simulink library "ddm"  (R2021b)
settings: Solver=VariableStepAuto  StartTime=0.0  StopTime=10.0  RelTol=1e-3
undefined symbols (not defined in the file or in its folder): ADDM_FrTMTqDev_X_Nm, ADDM_RrTMTqDev_X_Nm, ENUM_ADASACCSTA_ERROR, ENUM_ADASACCSTA_OFF, ENUM_ADASACCSTA_STANDBY, ENUM_ALLOWMOV_ALLOWREADY, ENUM_APS, ENUM_BRKSTA_ERROR, ENUM_BRKSTA_OFF, ENUM_BRKSTA_ON, ENUM_BRKSW_INVALID, ENUM_BRKSW_OFF, ENUM_BRKSW_ON, ENUM_CHGPREACTERRSTA_OBCPRE, ENUM_DCDCFAULTSTA_ANYFAULTLV1, ENUM_DCDCFAULTSTA_ANYFAULTLV2, ENUM_DRIVETRAIN_AWD, ENUM_DRIVETRAIN_FWD, ENUM_DRIVETRAIN_RWD, ENUM_EDUDRTSTA_NORMAL, ENUM_EPBSTA_APPLIED, ENUM_EPBSTA_RELEASED, ENUM_GEARACTUALPOSN_INVALID, ENUM_GEARACTUALPOSN_P, ENUM_HVBATTREADYPRE_READY, ENUM_MCUWARN_LV0, ENUM_MCUWARN_LV1, ENUM_MCUWARN_LV2, ENUM_MCUWARN_LV3, ENUM_MCUWARN_NOERROR, ENUM_OBCFAULTSTA_ANYFAULT, ENUM_PAS_R2F2, ENUM_PDFAULT_BATTPDFAIL, ENUM_PDFAULT_DCDCDISABLE, ENUM_PDFAULT_MCUDISABLE, ENUM_PDFAULT_MCUDISCHRG, ENUM_POWERSTA_OFF, ENUM_POWERSTA_ON, ENUM_POWERSTA_READY, ENUM_POWERSTA_STANDBY, ENUM_PRESSINDI_LOW, ENUM_PUFAULT_BATTUPFAIL, ENUM_PUFAULT_DCDCENABLEFAIL, ENUM_PUFAULT_PRECHRGCHKFAIL, ENUM_PUFAULT_SAFETYCHKFAIL, ENUM_PUSTATE_COMPLETED, ENUM_PWRSTASW_OFF, ENUM_PWRSTASW_OFFA, ENUM_PWRSTASW_OFFCHVCHRG, ENUM_PWRSTASW_OFFCLVCHRG, ENUM_PWRSTASW_ON, ENUM_PWRSTASW_ONHVCHRG, ENUM_PWRSTASW_READY, ENUM_PWRSTASW_STANDBY, ENUM_SHIFTCOMMAND_P, ENUM_SHIFTERERRSTA_PBUTTONFAILURE, ENUM_VEHMALFUNLV_2ND, ENUM_VEHMALFUNLV_3RD, ENUM_VEHMALFUNLV_4TH, ENUM_VEHMALFUNLV_NORMAL ... (+459)
libraries: hcu_lib x521, $bdroot x5, simulink x3
(part 2 of 25)

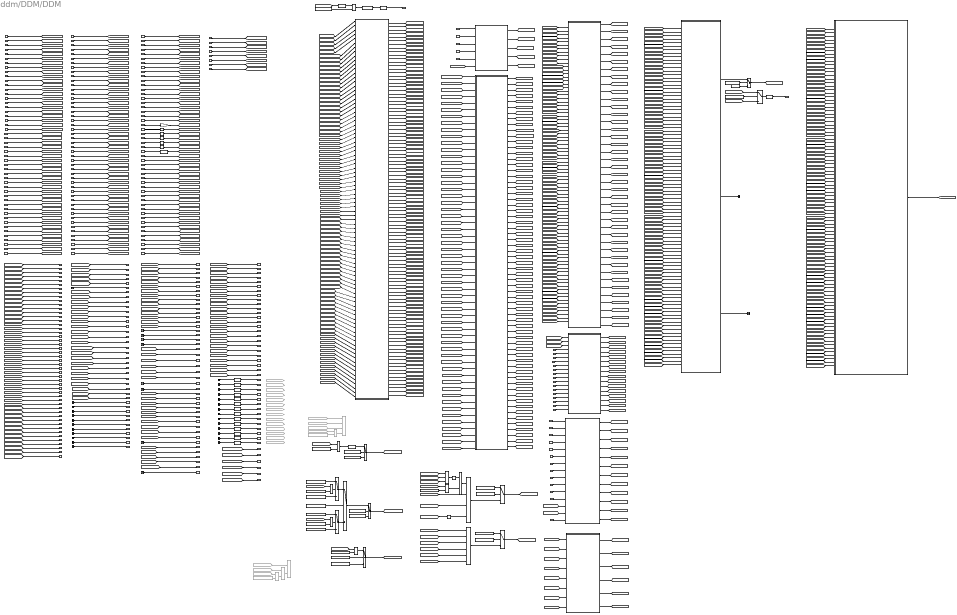
== system ddm/DDM/DDM ==
  note: RAPS Error signal
  note: EDriveSysErrVCUErr
  note: EDriveSysErrVCUErr
  note: Low battery system warning lamp
  task_time_s : Inport
  VINP_CANMsgValidABM1_flg : Inport  Port=2
  VINP_BrkPedalPosSta_enum : Inport  Port=3
  VINP_BrkPedalPos_pct : Inport  Port=4
  VINP_BrkSWSta_flg : Inport  Port=5
  VINP_CANMsgValidESC1_flg : Inport  Port=6
  VINP_CANMsgValidESC5_flg : Inport  Port=7
  VINP_VehSpeed_kph : Inport  Port=8
  VDDM_ESC1RCErr_flg : Inport  Port=9
  VDDM_ESC1CSErr_flg : Inport  Port=10
  VDDM_ESC5RCErr_flg : Inport  Port=11
  VDDM_ESC5CSErr_flg : Inport  Port=12
  VDDM_C1ABM1RCChk_flg : Inport  Port=13
  VDDM_C1ABM1CSChk_flg : Inport  Port=14
  VINP_EPBSta_enum : Inport  Port=15
  VINP_EPBErrSta_enum : Inport  Port=16
  VINP_EBDFailed_flg : Inport  Port=17
  VINP_HDDFailed_flg : Inport  Port=18
  VINP_ABSFailed_flg : Inport  Port=19
  VINP_TCSFailed_flg : Inport  Port=20
  VINP_ESCFailed_flg : Inport  Port=21
  VINP_HBBFailed_flg : Inport  Port=22
  VINP_PBAFailed_flg : Inport  Port=23
  VINP_HSAFailed_flg : Inport  Port=24
  VINP_AVHFailed_flg : Inport  Port=25
  VINP_MCPressureV_flg : Inport  Port=26
  VINP_BrkSwV_flg : Inport  Port=27
  VINP_BrkPedalPosSta_flg : Inport  Port=28
  VINP_LongAccelV_flg : Inport  Port=29
  VINP_LatAccelV_flg : Inport  Port=30
  VINP_YawRateV_flg : Inport  Port=31
  VINP_RFPulseCountV_flg : Inport  Port=32
  VINP_RRPulseCountV_flg : Inport  Port=33
  VINP_LFPulseCountV_flg : Inport  Port=34
  VINP_LRPulseCountV_flg : Inport  Port=35
  VINP_LRRawWhlSpeedV_flg : Inport  Port=36
  VINP_RRRawWhlSpeedV_flg : Inport  Port=37
  VINP_LFRawWhlSpeedV_flg : Inport  Port=38
  VINP_RFRawWhlSpeedV_flg : Inport  Port=39
  VINP_CANMsgValidEPS1_flg : Inport  Port=40
  VINP_SASV_flg : Inport  Port=41
  VINP_CANMsgValidEPB1_flg : Inport  Port=42
  VDDM_EPB1RCErr_flg : Inport  Port=43
  VDDM_EPB1CSErr_flg : Inport  Port=44
  VDDM_EPSRCErr_flg : Inport  Port=45
  VDDM_EPSCSErr_flg : Inport  Port=46
  VINP_CANMsgValidBMS1_flg : Inport  Port=47
  VINP_CANMsgValidBMS6_flg : Inport  Port=48
  VINP_CANMsgValidCCU1_flg : Inport  Port=49
  VINP_CANMsgValidCCU2_flg : Inport  Port=50
  VINP_BMSWarn1_flg : Inport  Port=51
  VINP_BMSWarn2_flg : Inport  Port=52
  VINP_BMSWarn3_flg : Inport  Port=53
  VINP_BMSWarn4_flg : Inport  Port=54
  VINP_BMSWarn5_flg : Inport  Port=55
  VINP_BMSWarn6_flg : Inport  Port=56
  VINP_BMSWarn7_flg : Inport  Port=57
  VINP_BMSWarn8_flg : Inport  Port=58
  VINP_DCDCFaultSta_enum : Inport  Port=59
  VINP_OBCFaultSta_enum : Inport  Port=60
  VINP_MCUWarnFNidec_enum : Inport  Port=61
  VINP_MCUWarnRNidec_enum : Inport  Port=62
  VINP_LVBattDet12V_V : Inport  Port=63
  VINP_BMSREADY_flg : Inport  Port=64
  VINP_HVBattReady4Pre_enum : Inport  Port=65
  VINP_HVBContactorSta_flg : Inport  Port=66
  VINP_DCDCReady4Pre_flg : Inport  Port=67
  VINP_DCDCEnabled_flg : Inport  Port=68
  VINP_CANMsgValidMCUNF1_flg : Inport  Port=69
  VINP_CANMsgValidMCUNR1_flg : Inport  Port=70
  VINP_CANMsgValidShifter1_flg : Inport  Port=71
  VINP_FrEDUDrtStaNidec_flg : Inport  Port=72
  VINP_FrEDURealTMTqNidec_Nm : Inport  Port=73
  VINP_RrEDUDrtStaNidec_flg : Inport  Port=74
  VINP_RrEDURealTMTqNidec_Nm : Inport  Port=75
  VDDM_C3BMS6RCChk_flg : Inport  Port=76
  VDDM_C3BMS6CSChk_flg : Inport  Port=77
  VDDM_C3BMS1RCChk_flg : Inport  Port=78
  VDDM_C3BMS1CSChk_flg : Inport  Port=79
  VDDM_C3CCU1RCChk_flg : Inport  Port=80
  VDDM_C3CCU1CSChk_flg : Inport  Port=81
  VDDM_C3CCU2RCChk_flg : Inport  Port=82
  VDDM_C3CCU2CSChk_flg : Inport  Port=83
  VDDM_MCUNF1RCErr_flg : Inport  Port=84
  VDDM_MCUNF1CSErr_flg : Inport  Port=85
  VDDM_MCUNR1RCErr_flg : Inport  Port=86
  VDDM_MCUNR1CSErr_flg : Inport  Port=87
  VDDM_Shifter1RCErr_flg : Inport  Port=88
  VDDM_Shifter1CSErr_flg : Inport  Port=89
  VINP_HVBattSOC_pct : Inport  Port=90
  VINP_ShifterHandleCmd_enum : Inport  Port=91
  VINP_ShifterFailsta_enum : Inport  Port=92
  VINP_CANMsgValidBMS5_flg : Inport  Port=93
  VPMM_PowerSta_enum : Inport  Port=94
  VPMM_PwrStaSW_enum : Inport  Port=95
  VPMM_PowerUpFault_enum : Inport  Port=96
  VPMM_PowerDownFault_enum : Inport  Port=97
  VPMM_DrivetrainSelect_enum : Inport  Port=98
  VPMM_SafetyChkHLv_flg : Inport  Port=99
  VPMM_SafetyChkMLv_flg : Inport  Port=100
  VPMM_HVChrgPreActionErrSta_enum : Inport  Port=101
  VPMM_MCUReady_flg : Inport  Port=102
  VPMM_MCUReady4Pre_flg : Inport  Port=103
  VPMM_PowerUpState_enum : Inport  Port=104
  VPMM_MCUDCBusMaxVolt_V : Inport  Port=105
  VINP_BrakeSWGPIO_flg : Inport  Port=106
  VINP_BrakeLampSW_flg : Inport  Port=107
  VINP_DrStSW : Inport  Port=108
  VINP_FLAJARSW : Inport  Port=109
  VINP_FRAJARSW : Inport  Port=110
  VINP_RLAJARSW : Inport  Port=111
  VINP_RRAJARSW : Inport  Port=112
  VINP_HoodSW : Inport  Port=113
  VINP_TailgaSW : Inport  Port=114
  VINP_AccelPedal1Vol_V : Inport  Port=115
  VINP_AccelPedal2Vol_V : Inport  Port=116
  VDKC_DKCAuthSta_enum : Inport  Port=117
  VINP_AllowMovThd_OTA_enum : Inport  Port=118
  VINP_Pedal1Ref5V_V : Inport  Port=119
  VINP_Pedal2Ref5V_V : Inport  Port=120
  VINP_AuxBattVolmV_mV : Inport  Port=121
  VINP_CAN1BusOff_flg : Inport  Port=122
  VINP_CAN3BusOff_flg : Inport  Port=123
  VINP_CAN4BusOff_flg : Inport  Port=124
  VINP_CAN6BusOff_flg : Inport  Port=125
  VINP_CAN1BusError_flg : Inport  Port=126
  VINP_CAN2BusError_flg : Inport  Port=127
  VINP_CAN3BusError_flg : Inport  Port=128
  VINP_CAN4BusError_flg : Inport  Port=129
  VINP_CAN5BusError_flg : Inport  Port=130
  VINP_CAN6BusError_flg : Inport  Port=131
  No_CAN_BUS_OFF : Inport  Port=132
  DTC_clear_request : Inport  Port=133
  VDHP_EAPCRBAD_flg : Inport  Port=134
  VDHP_EAPS1BAD_flg : Inport  Port=135
  VDHP_EAPS2BAD_flg : Inport  Port=136
  VDHP_EAPS12RangeSta_enum : Inport  Port=137
  VBCM_DiagHCrash_flg : Inport  Port=138
  VBCM_DiagFLTS_flg : Inport  Port=139
  VBCM_DiagFRTS_flg : Inport  Port=140
  VBCM_DiagRLTS_flg : Inport  Port=141
  VBCM_DiagRRTS_flg : Inport  Port=142
  VAPM_USSStaFCL_flg : Inport  Port=143
  VAPM_USSStaFML_flg : Inport  Port=144
  VAPM_USSStaFMR_flg : Inport  Port=145
  VAPM_USSStaFCR_flg : Inport  Port=146
  VAPM_USSStaRCL_flg : Inport  Port=147
  VAPM_USSStaRML_flg : Inport  Port=148
  VAPM_USSStaRMR_flg : Inport  Port=149
  VAPM_USSStaRCR_flg : Inport  Port=150
  VAPM_USSStaFLL_flg : Inport  Port=151
  VAPM_USSStaFLR_flg : Inport  Port=152
  VAPM_USSStaRLL_flg : Inport  Port=153
  VAPM_USSStaRLR_flg : Inport  Port=154
  VAPM_SNSRLayout_enum : Inport  Port=155
  VINP_DrStdAErrSta_enum : Inport  Port=156
  VINP_ZoneDrMalfunLevel_enum : Inport  Port=157
  VINP_CANMsgValidZoneDrVCU_flg : Inport  Port=158
  VINP_CANMsgValidZoneFrVCU_flg : Inport  Port=159
  VINP_CANMsgValidDKC1_flg : Inport  Port=160
  VINP_CANMsgValidDKC2_flg : Inport  Port=161
  ZoneFrMalfunLevel_enum : Inport  Port=162
  VVMC_ADASActive_flg : Inport  Port=163
  VVMC_APSActive_flg : Inport  Port=164
  VTQR_FrTMTqReq_Nm : Inport  Port=165
  VTQR_RrTMTqReq_Nm : Inport  Port=166
  VTPM_LFBatwarn_flg : Inport  Port=167
  VTPM_RFBatwarn_flg : Inport  Port=168
  VTPM_LRBatwarn_flg : Inport  Port=169
  VTPM_RRBatwarn_flg : Inport  Port=170
  VTPM_LFPressIndi_enum : Inport  Port=171
  VTPM_RFPressIndi_enum : Inport  Port=172
  VTPM_LRPressIndi_enum : Inport  Port=173
  VTPM_RRPressIndi_enum : Inport  Port=174
  VTPM_LFWheelTmpIndi_flg : Inport  Port=175
  VTPM_RFWheelTmpIndi_flg : Inport  Port=176
  VTPM_LRWheelTmpIndi_flg : Inport  Port=177
  VTPM_RRWheelTmpIndi_flg : Inport  Port=178
  VTPM_LFSensorFail_flg : Inport  Port=179
  VTPM_RFSensorFail_flg : Inport  Port=180
  VTPM_LRSensorFail_flg : Inport  Port=181
  VTPM_RRSensorFail_flg : Inport  Port=182
  VTQD_ActParkRequest_flg : Inport  Port=183
  VINP_ZoneSpdCtrlMode_enum : Inport  Port=184
  VTQD_GearActualPosn_enum : Inport  Port=185
  VTQD_ExternalTqAllow_flg : Inport  Port=186
  VTQD_ExtDoorAllow_flg : Inport  Port=187
  VINP_CANMsgValidFCM1_flg : Inport  Port=188
  VDDM_FCM1RCErr_flg : Inport  Port=189
  VDDM_FCM1CSErr_flg : Inport  Port=190
  VINP_ADASACCSta_enum : Inport  Port=191
  VINP_ACCRequireAccel_mps2 : Inport  Port=192
  APM : Subsystem
  BCM : Subsystem
  Chart : Stateflow chart  TreatAsAtomicUnit=on
      settings: PortSchema="{\"entries\":[{\"content\":{\"sides\":[{\"content\":{\"connectorIds\":[]},\"type\":\"ConnectorPlacement.EquallySpacedRectSide\",\"uuid\":\"5c49d68c-3a13-4722-ae51-60c531d65ae1\"},{\"content\":{\"connectorIds\":[],\"side\":\"RIGHT\"},\"type\":\"ConnectorPlacement.EquallySpacedRectSide\",\"uuid\":\"1499f12d-58db-4e43-953b-81e532540c9e\"},{\"content\":{\"connectorIds\":[\"Out1\",\"Out2\",\"Out3\"],\"side\":\"TOP\"},\"type\":\"ConnectorPlacement.EquallySpacedRectSide\",\"uuid\":\"b40fb5a5-59a6-496c-b268-75370edec7d4\"},{\"content\":{\"connectorIds\":[\"In2\",\"In3\",\"In4\",\"In5\",\"In6\",\"In7\",\"In8\",\"In9\",\"In10\",\"In11\",\"In12\",\"In13\",\"In14\",\"In15\",\"In16\",\"In17\",\"In18\",\"In19\",\"In20\",\"In21\",\"In22\",\"In23\",\"In24\",\"In25\",\"In26\",\"In27\",\"In28\",\"In29\",\"In30\",\"In31\",\"In32\",\"In33\",\"In34\",\"In35\",\"In36\",\"In37\",\"In38\",\"In39\",\"In40\",\"In41\",\"In42\",\"In43\",\"In44\",\"In45\",\"In46\",\"In47\",\"In1\",\"In48\",\"In49\",\"In50\",\"In51\",\"In52\",\"In53\",\"In54\",\"In55\",\"In56\",\"In57\",\"In58\",\"In59\",\"In60\",\"In61\",\"In62\",\"In63\",\"In64\",\"In65\",\"In66\",\"In67\",\"In68\",\"In69\",\"In70\",\"In71\",\"In72\",\"In73\",\"In74\",\"In75\",\"In76\",\"In77\",\"In78\",\"In79\",\"In80\",\"In81\",\"In82\",\"In83\",\"In84\",\"In85\",\"In86\",\"In87\",\"In88\",\"In89\",\"In90\",\"In91\",\"In92\",\"In93\",\"In94\",\"In95\",\"In96\"],\"side\":\"BOTTOM\"},\"type\":\"ConnectorPlacement.EquallySpacedRectSide\",\"uuid\":\"7a3e18bf-6f06-4df1-889c-341cd16aa4bd\"}]},\"type\":\"ConnectorPlacement.EquallySpacedConnector\",\"uuid\":\"c096d691-37a2-471f-9d84-793135a13589\"}],\"packageUris\":[\"http://schema.mathworks.com/mf0/Connector/R2020b\"],\"version\":\"1.0\"}"
  Constant : Constant  Value=ENUM_PWRSTASW_READY
  Constant1 : Constant  Value=ZERO_INT
  Constant10 : Constant  Value=KDDM_VCURAPSErrLv2_flg_ovrdval
  Constant11 : Constant  Commented=on  Value=ENUM_VEHMALFUNLV_2ND
  Constant12 : Constant  Value=ENUM_VEHMALFUNLV_2ND
  Constant13 : Constant  Value=KDDM_DiagnosisTmp_flg_ovrdflg
  Constant14 : Constant  Value=KDDM_VCURAPSErrLv2_flg_ovrdflg
  Constant15 : Constant  Value=KDDM_VehMalfunLevelSW_flg
  Constant16 : Constant  Value=ENUM_DCDCFAULTSTA_ANYFAULTLV2
  Constant17 : Constant  Value=ENUM_VEHMALFUNLV_3RD
  Constant18 : Constant  Value=KDDM_SysErrVCUErrSW_flg
  Constant19 : Constant  Value=KDDM_LimpHomeTmpSW_flg
  Constant{2,5,21..22,24} (5 alike) : Constant  Value=FALSE
  Constant20 : Constant  Value=ENUM_VEHMALFUNLV_2ND
  Constant23 : Constant  Value=KDDM_SysErrPwrOutSW_flg
  Constant3 : Constant  Value=TRUE
  Constant36 : Constant  Commented=on  Value=ENUM_DCDCFAULTSTA_ANYFAULTLV2
  Constant4 : Constant  Value=KDDM_DiagnosisTmp_flg_ovrdflg
  Constant6 : Constant  Value=KDDM_VCURAPSErrLv3_flg_ovrdval
  Constant7 : Constant  Value=ENUM_VEHMALFUNLV_2ND
  Constant8 : Constant  Value=TRUE
  Constant9 : Constant  Value=KDDM_VCURAPSErrLv3_flg_ovrdflg
  Data Type Conversion{,2..14,56} (15 alike) : DataTypeConversion  OutDataTypeStr=boolean
  Data Type Conversion1 : DataTypeConversion
  Data Type Conversion15 : DataTypeConversion  OutDataTypeStr=uint8
  Data Type Conversion49 : DataTypeConversion  OutDataTypeStr=uint8
  Detect Increase : simulink/Logic and Bit Operations/Detect Increase  vinit=0.0  OutDataTypeStr=boolean
  Enabled Subsystem : Subsystem  TreatAsAtomicUnit=on
  Equal : RelationalOperator  Operator===  OutDataTypeStr=boolean  RndMeth=Simplest
  Equal1 : RelationalOperator  Operator===  OutDataTypeStr=boolean  RndMeth=Simplest
  Equal14 : RelationalOperator  Commented=on  Operator===  OutDataTypeStr=boolean  RndMeth=Simplest
  From206 : From  Commented=on  GotoTag=VDDM_VehMalfunLevel_enum
  From514 : From  Commented=on  GotoTag=VDDM_EDriveSysErrTQD_flg
  From515 : From  Commented=on  GotoTag=VDDM_EDriveSysErrPMM_flg
  From516 : From  Commented=on  GotoTag=VDDM_EDriveSysErrVCUErrVMC_flg
  From530 : From  Commented=on  GotoTag=VDDM_SysAllowReadySta_flg
  From531 : From  Commented=on  GotoTag=VDDM_VCUFLDoorSta_flg
  From532 : From  Commented=on  GotoTag=VDDM_VCUFRDoorSta_flg
  From533 : From  Commented=on  GotoTag=VDDM_VCURLDoorSta_flg
  From534 : From  Commented=on  GotoTag=VDDM_VCURRDoorSta_flg
  From535 : From  Commented=on  GotoTag=VDDM_VCUHoodSWSta_flg
  From536 : From  Commented=on  GotoTag=VDDM_VCUTailgateSWSta_flg
  From537 : From  Commented=on  GotoTag=VDDM_VCUBrkSWSta_enum
  From538 : From  Commented=on  GotoTag=VDDM_Lv2ErrCFS_flg
  From539 : From  Commented=on  GotoTag=VDDM_MCUActDisFail_flg
  From540 : From  Commented=on  GotoTag=VDDM_HVRlyOpFail_flg
  From541 : From  Commented=on  GotoTag=VDDM_EPB1NoComCFS_flg
  From594 : From  Commented=on  GotoTag=VDDM_PMMBattErr_flg
  From595 : From  Commented=on  GotoTag=VINP_DCDCFaultSta_enum
  From601 : From  Commented=on  GotoTag=VDDM_EPB1RCErrCFS_flg
  From602 : From  Commented=on  GotoTag=VDDM_EPB1CSErrCFS_flg
  From603 : From  Commented=on  GotoTag=VDDM_EPBSigErrCFS_flg
  Gain : Gain  Gain=XX2KXX
  Ground{,1..2,4..32,35..36} (34 alike) : Ground
  Latch : hcu_lib/Basic_Blocks/Latch
  Logical Operator : Logic  Operator=OR  Inputs=4  AllPortsSameDT=off  OutDataTypeStr=boolean
  Logical Operator1 : Logic  Commented=on  Operator=OR  Inputs=4  AllPortsSameDT=off  OutDataTypeStr=boolean
  Logical Operator{3,6..7,10..13} (7 alike) : Logic  Operator=NOT  AllPortsSameDT=off  OutDataTypeStr=boolean
  Logical Operator2 : Logic  Operator=OR  Inputs=6  AllPortsSameDT=off  OutDataTypeStr=boolean
  Logical Operator4 : Logic  Commented=on  Operator=OR  AllPortsSameDT=off  OutDataTypeStr=boolean
  Logical Operator5 : Logic  Commented=on  Operator=OR  AllPortsSameDT=off  OutDataTypeStr=boolean
  Logical Operator8 : Logic  AllPortsSameDT=off  OutDataTypeStr=boolean
  Logical Operator9 : Logic  Operator=OR  Inputs=3  AllPortsSameDT=off  OutDataTypeStr=boolean
  PMM : Subsystem
  Relational Operator{,1,3..4} (4 alike) : RelationalOperator  OutDataTypeStr=boolean  RndMeth=Simplest
  Relational Operator2 : RelationalOperator  Commented=on  OutDataTypeStr=boolean  RndMeth=Simplest
  Subsystem : Subsystem
  Switch{,7..9} (4 alike) : Switch  Criteria=u2 > Threshold
  Switch{1..6} (6 alike) : Switch  Criteria=u2 ~= 0
  TPM : Subsystem
  TQD : Subsystem
  Terminator : Terminator
  Terminator1 : Terminator
  VMC_DDM : Subsystem
  VDDM_C3BMS6RCDTC_raw32 : Outport
  VDDM_C3BMS6CSDTC_raw32 : Outport  Port=2
  VDDM_C3BMS6LCDTC_raw32 : Outport  Port=3
  VDDM_C3BMS1RCDTC_raw32 : Outport  Port=4
  VDDM_C3BMS1CSDTC_raw32 : Outport  Port=5
  VDDM_C3BMS1LCDTC_raw32 : Outport  Port=6
  VDDM_C3CCU1RCDTC_raw32 : Outport  Port=7
  VDDM_C3CCU1CSDTC_raw32 : Outport  Port=8
  VDDM_C3CCU1LCDTC_raw32 : Outport  Port=9
  VDDM_C3CCU2RCDTC_raw32 : Outport  Port=10
  VDDM_C3CCU2CSDTC_raw32 : Outport  Port=11
  VDDM_C3CCU2LCDTC_raw32 : Outport  Port=12
  VDDM_C1ABM1RCDTC_raw32 : Outport  Port=13
  VDDM_C1ABM1CSDTC_raw32 : Outport  Port=14
  VDDM_C1ABM1LCDTC_raw32 : Outport  Port=15
  VDDM_Lv1ErrDTC_raw32 : Outport  Port=16
  VDDM_Lv2ErrDTC_raw32 : Outport  Port=17
  VDDM_Lv3ErrDTC_raw32 : Outport  Port=18
  VDDM_Lv4ErrDTC_raw32 : Outport  Port=19
  VDDM_BrkSWErrDTC_raw32 : Outport  Port=20
  VDDM_BrkSWNoBacDTC_raw32 : Outport  Port=21
  VDDM_KeyAuthDTC_raw32 : Outport  Port=22
  VDDM_ONtoRdyDTC_raw32 : Outport  Port=23
  VDDM_HVB4PreDTC_raw32 : Outport  Port=24
  VDDM_MCU4PreDTC_raw32 : Outport  Port=25
  VDDM_DCDC4PreDTC_raw32 : Outport  Port=26
  VDDM_HVRlyCloDTC_raw32 : Outport  Port=27
  VDDM_BMSRdyDTC_raw32 : Outport  Port=28
  VDDM_DCDCEnaDTC_raw32 : Outport  Port=29
  VDDM_HiLvSaChkDTC_raw32 : Outport  Port=30
  VDDM_MidLvSaChkDTC_raw32 : Outport  Port=31
  VDDM_MCUDisDTC_raw32 : Outport  Port=32
  VDDM_DCDCDisDTC_raw32 : Outport  Port=33
  VDDM_HVRlyOpDTC_raw32 : Outport  Port=34
  VDDM_MCUActDTC_raw32 : Outport  Port=35
  VDDM_OBC4PreDTC_raw32 : Outport  Port=36
  VDDM_IniLVLoDTC_raw32 : Outport  Port=37
  VDDM_LVSupLoDTC_raw32 : Outport  Port=38
  VDDM_LVSupHiDTC_raw32 : Outport  Port=39
  VDDM_LVInErrDTC_raw32 : Outport  Port=40
  VDDM_DrStSWDTC_raw32 : Outport  Port=41
  VDDM_FLDoorSWDTC_raw32 : Outport  Port=42
  VDDM_RLDoorSWDTC_raw32 : Outport  Port=43
  VDDM_FRDoorSWDTC_raw32 : Outport  Port=44
  VDDM_RRDoorSWDTC_raw32 : Outport  Port=45
  VDDM_HoodSWDTC_raw32 : Outport  Port=46
  VDDM_TailgaSWDTC_raw32 : Outport  Port=47
  VDDM_EDriveSysErrVCUErr_flg : Outport  Port=48
  VDDM_VehMalfunLevel_enum : Outport  Port=49
  VDDM_APS1SigOoRDTC_raw32 : Outport  Port=50
  VDDM_APS2SigOoRDTC_raw32 : Outport  Port=51
  VDDM_APSCorrErrDTC_raw32 : Outport  Port=52
  VDDM_MCUF1NoComDTC_raw32 : Outport  Port=53
  VDDM_MCUR1NoComDTC_raw32 : Outport  Port=54
  VDDM_Shifter1NoComDTC_raw32 : Outport  Port=55
  VDDM_ESC7NoComDTC_raw32 : Outport  Port=56
  VDDM_ESC1NoComDTC_raw32 : Outport  Port=57
  VDDM_ESC5NoComDTC_raw32 : Outport  Port=58
  VDDM_EnterNewOperCyc_flg : Outport  Port=59
  VDDM_DiagHCrashDTC_raw32 : Outport  Port=60
  VDDM_DiagFLTSDTC_raw32 : Outport  Port=61
  VDDM_DiagFRTSDTC_raw32 : Outport  Port=62
  VDDM_DiagRLTSDTC_raw32 : Outport  Port=63
  VDDM_DiagRRTSDTC_raw32 : Outport  Port=64
  VDDM_FCLUSSDTC_raw32 : Outport  Port=65
  VDDM_FMLUSSDTC_raw32 : Outport  Port=66
  VDDM_FMRUSSDTC_raw32 : Outport  Port=67
  VDDM_FCRUSSDTC_raw32 : Outport  Port=68
  VDDM_RCLUSSDTC_raw32 : Outport  Port=69
  VDDM_RMLUSSDTC_raw32 : Outport  Port=70
  VDDM_RMRUSSDTC_raw32 : Outport  Port=71
  VDDM_RCRUSSDTC_raw32 : Outport  Port=72
  VDDM_FLLUSSDTC_raw32 : Outport  Port=73
  VDDM_FLRUSSDTC_raw32 : Outport  Port=74
  VDDM_RLLUSSDTC_raw32 : Outport  Port=75
  VDDM_RLRUSSDTC_raw32 : Outport  Port=76
  VDDM_FCM2NoComDTC_raw32 : Outport  Port=77
  VDDM_FCM2RCErrDTC_raw32 : Outport  Port=78
  VDDM_FCM2CSErrDTC_raw32 : Outport  Port=79
  VDDM_FCM3NoComDTC_raw32 : Outport  Port=80
  VDDM_FCM3RCErrDTC_raw32 : Outport  Port=81
  VDDM_FCM3CSErrDTC_raw32 : Outport  Port=82
  VDDM_FCM4NoComDTC_raw32 : Outport  Port=83
  VDDM_FCM4CSErrDTC_raw32 : Outport  Port=84
  VDDM_FCM5NoComDTC_raw32 : Outport  Port=85
  VDDM_FCM5CSErrDTC_raw32 : Outport  Port=86
  VDDM_ZoneSCPNoComDTC_raw32 : Outport  Port=87
  VDDM_BMSSigErrDetDTC_raw32 : Outport  Port=88
  VDDM_FCMACCSigErrDetDTC_raw32 : Outport  Port=89
  VDDM_FrMCUSigErrDetDTC_raw32 : Outport  Port=90
  VDDM_RrMCUSigErrDetDTC_raw32 : Outport  Port=91
  VDDM_CCUSigErrDetDTC_raw32 : Outport  Port=92
  VDDM_ACCAccelCmdErrDetDTC_raw32 : Outport  Port=93
  VDDM_ACCMalfuncDetDTC_raw32 : Outport  Port=94
  VDDM_CCMalfuncDetDTC_raw32 : Outport  Port=95
  VDDM_MSAMalfuncDetDTC_raw32 : Outport  Port=96
  VDDM_ISAMalfuncDetDTC_raw32 : Outport  Port=97
  VDDM_MCUF1RCErrDTC_raw32 : Outport  Port=98
  VDDM_MCUR1RCErrDTC_raw32 : Outport  Port=99
  VDDM_MCUF1CSErrDTC_raw32 : Outport  Port=100
  VDDM_MCUR1CSErrDTC_raw32 : Outport  Port=101
  VDDM_Shifter1RCErrDTC_raw32 : Outport  Port=102
  VDDM_Shifter1CSErrDTC_raw32 : Outport  Port=103
  VDDM_ESC7RCErrDTC_raw32 : Outport  Port=104
  VDDM_ESC7CSErrDTC_raw32 : Outport  Port=105
  VDDM_ESC1RCErrDTC_raw32 : Outport  Port=106
  VDDM_ESC1CSErrDTC_raw32 : Outport  Port=107
  VDDM_ESC5RCErrDTC_raw32 : Outport  Port=108
  VDDM_ESC5C  SErrDTC_raw32 : Outport  Port=109
  VDDM_FrMCUTqErrDTC_raw32 : Outport  Port=110
  VDDM_RrMCUTqErrDTC_raw32 : Outport  Port=111
  VDDM_LFBatwarnDTC_raw32 : Outport  Port=112
  VDDM_RFBatwarnDTC_raw32 : Outport  Port=113
  VDDM_LRBatwarnDTC_raw32 : Outport  Port=114
  VDDM_RRBatwarnDTC_raw32 : Outport  Port=115
  VDDM_LFPressIndiDTC_raw32 : Outport  Port=116
  VDDM_RFPressIndiDTC_raw32 : Outport  Port=117
  VDDM_LRPressIndiDTC_raw32 : Outport  Port=118
  VDDM_RRPressIndiDTC_raw32 : Outport  Port=119
  VDDM_LFWheelTmpHighDTC_raw32 : Outport  Port=120
  VDDM_RFWheelTmpHighDTC_raw32 : Outport  Port=121
  VDDM_LRWheelTmpHighDTC_raw32 : Outport  Port=122
  VDDM_RRWheelTmpHighDTC_raw32 : Outport  Port=123
  VDDM_LFSensorFailDTC_raw32 : Outport  Port=124
  VDDM_RFSensorFailDTC_raw32 : Outport  Port=125
  VDDM_LRSensorFailDTC_raw32 : Outport  Port=126
  VDDM_RRSensorFailDTC_raw32 : Outport  Port=127
  VDDM_C1EPAS2LCDTC_raw32 : Outport  Port=128
  VDDM_5vAPS1PwrErrDTC_raw32 : Outport  Port=129
  VDDM_5vAPS2PwrErrDTC_raw32 : Outport  Port=130
  VDDM_EPBLockTODTC_raw32 : Outport  Port=131
  VDDM_EPBUnlockTODTC_raw32 : Outport  Port=132
  VDDM_LimpHomeActTmp_flg : Outport  Port=133
  VDDM_EDriveSysErr_VCUErrTmp_flg : Outport  Port=134
  VDDM_EPB1NoComDTC_raw32 : Outport  Port=135
  VDDM_EPB1RCErrDTC_raw32 : Outport  Port=136
  VDDM_EPB1CSErrDTC_raw32 : Outport  Port=137
  VDDM_EPBSigErrDTC_raw32 : Outport  Port=138
  VDDM_FCM1NoComDTC_raw32 : Outport  Port=139
  VDDM_FCM1RCErrDTC_raw32 : Outport  Port=140
  VDDM_FCM1CSErrDTC_raw32 : Outport  Port=141
  VDDM_ESCSigErrDetDTC_raw32 : Outport  Port=142
  VDDM_ShifterSigErrDetDTC_raw32 : Outport  Port=143
  VDDM_DrVCUNoComDTC_raw32 : Outport  Port=144
  VDDM_FrVCUNoComDTC_raw32 : Outport  Port=145
  VDDM_ZoneDrSigErrDetDTC_raw32 : Outport  Port=146
  VDDM_ZoneFrSigErrDetDTC_raw32 : Outport  Port=147
  VDDM_EPS1NoComDTC_raw32 : Outport  Port=148
  VDDM_EPS1RCErrDTC_raw32 : Outport  Port=149
  VDDM_EPS1CSErrDTC_raw32 : Outport  Port=150
  VDDM_EPSSigErrDTC_raw32 : Outport  Port=151
  VDDM_DTCDetect_enum : Outport  Port=152
  VDDM_EngagePFail_flg : Outport  Port=153
  VDDM_DisengagePFail_flg : Outport  Port=154
  VDDM_VCURAPSErrLv2_flg : Outport  Port=155
  VDDM_VCURAPSErrLv3_flg : Outport  Port=156
  VDDM_EDriveSysErrShifterErr_flg : Outport  Port=157
  VDDM_PMMBattErr_flg : Outport  Port=158
  VDDM_LVSysErrPwrOutErr_flg : Outport  Port=159
  VDDM_HVRlyOpFail_flg : Outport  Port=160
  VDDM_MCUActDisFail_flg : Outport  Port=161
  VDDM_VCUBrkSWSta_enum : Outport  Port=162
  VDDM_VCUFLDoorSta_flg : Outport  Port=163
  VDDM_VCUFRDoorSta_flg : Outport  Port=164
  VDDM_VCURLDoorSta_flg : Outport  Port=165
  VDDM_VCURRDoorSta_flg : Outport  Port=166
  VDDM_SysAllowReadySta_flg : Outport  Port=167
  VDDM_VCUHoodSWSta_flg : Outport  Port=168
  VDDM_VCUTailgateSWSta_flg : Outport  Port=169
  VDDM_EPB1NoComCFS_flg : Outport  Port=170
  VDDM_EPB1RCErrCFS_flg : Outport  Port=171
  VDDM_EPB1CSErrCFS_flg : Outport  Port=172
  VDDM_EPBSigErrCFS_flg : Outport  Port=173
  VDDM_CAN1BusErrorDTC_raw32 : Outport  Port=174
  VDDM_CAN2BusErrorDTC_raw32 : Outport  Port=175
  VDDM_CAN3BusErrorDTC_raw32 : Outport  Port=176
  VDDM_CAN4BusErrorDTC_raw32 : Outport  Port=177
  VDDM_CAN5BusErrorDTC_raw32 : Outport  Port=178
  VDDM_CAN6BusErrorDTC_raw32 : Outport  Port=179
  wires:
  VINP_ZoneDrMalfunLevel_enum/1 -> [VINP_ZoneDrMalfunLevel_enum]
  PMM/56(VDDM_SysAllowReadySta_flg) -> [VDDM_SysAllowReadySta_flg]
  PMM/55(VDDM_VCUBrkSWSta_enum) -> [VDDM_VCUBrkSWSta_enum]
  [VDDM_EPBUnlockTODTC_raw32] -> VDDM_EPBUnlockTODTC_raw32/1
  [VDDM_EPBLockTODTC_raw32] -> VDDM_EPBLockTODTC_raw32/1
  [VDDM_EPBUnlockTOCFS_flg] -> Chart/27(VDDM_EPBUnlockTOCFS_flg)
  [VDDM_EPBLockTOCFS_flg] -> Chart/26(VDDM_EPBLockTOCFS_flg)
  VINP_ShifterHandleCmd_enum/1 -> [VINP_ShifterHandleCmd_enum]
  VINP_EPBSta_enum/1 -> [VINP_EPBSta_enum]
  VTQD_ActParkRequest_flg/1 -> [VTQD_ActParkRequest_flg]
  [VINP_ShifterHandleCmd_enum] -> TQD/40(VINP_ShifterHandleCmd_enum)
  [VINP_EPBSta_enum] -> TQD/39(VINP_EPBSta_enum)
  [VTQD_ActParkRequest_flg] -> TQD/38(VTQD_ActParkRequest_flg)
  [VDDM_AuxBattVolV_V] -> TQD/37(VDDM_AuxBattVolV_V)
  Gain/1 -> [VDDM_AuxBattVolV_V]
  VINP_AuxBattVolmV_mV/1 -> Gain/1
  [VDDM_5vAPS2PwrErrDTC_raw32] -> VDDM_5vAPS2PwrErrDTC_raw32/1
  [VDDM_5vAPS1PwrErrDTC_raw32] -> VDDM_5vAPS1PwrErrDTC_raw32/1
  TQD/34(VDDM_5vAPS2OoRDTC_raw32) -> [VDDM_5vAPS2PwrErrDTC_raw32]
  TQD/33(VDDM_5vAPS1OoRDTC_raw32) -> [VDDM_5vAPS1PwrErrDTC_raw32]
  [VINP_HVBattSOC_pct] -> TQD/36(VINP_HVBattSOC_pct)
  VINP_HVBattSOC_pct/1 -> [VINP_HVBattSOC_pct]
  [VINP_Pedal2Ref5V_V] -> TQD/35(VINP_Pedal2Ref5V_V)
  [VINP_Pedal1Ref5V_V] -> TQD/34(VINP_Pedal1Ref5V_V)
  VINP_Pedal2Ref5V_V/1 -> [VINP_Pedal2Ref5V_V]
  VINP_Pedal1Ref5V_V/1 -> [VINP_Pedal1Ref5V_V]
  [VDDM_RRSensorFailDTC_raw32] -> VDDM_RRSensorFailDTC_raw32/1
  [VDDM_LRSensorFailDTC_raw32] -> VDDM_LRSensorFailDTC_raw32/1
  [VDDM_RFSensorFailDTC_raw32] -> VDDM_RFSensorFailDTC_raw32/1
  [VDDM_LFSensorFailDTC_raw32] -> VDDM_LFSensorFailDTC_raw32/1
  TPM/15(VDDM_LRSensorFailDTC_raw32) -> [VDDM_LRSensorFailDTC_raw32]
  TPM/14(VDDM_RFSensorFailDTC_raw32) -> [VDDM_RFSensorFailDTC_raw32]
  TPM/16(VDDM_RRSensorFailDTC_raw32) -> [VDDM_RRSensorFailDTC_raw32]
  TPM/13(VDDM_LFSensorFailDTC_raw32) -> [VDDM_LFSensorFailDTC_raw32]
  VTPM_LFSensorFail_flg/1 -> TPM/16(VTPM_LFSensorFail_flg)
  VTPM_RFSensorFail_flg/1 -> TPM/17(VTPM_RFSensorFail_flg)
  VTPM_LRSensorFail_flg/1 -> TPM/18(VTPM_LRSensorFail_flg)
  VTPM_RRSensorFail_flg/1 -> TPM/19(VTPM_RRSensorFail_flg)
  VAPM_SNSRLayout_enum/1 -> APM/15(VAPM_SNSRLayout_enum)
  Ground21/1 -> VDDM_C1EPAS2LCDTC_raw32/1  "VDDM_C1EPAS2LCDTC_raw32"
  [VDDM_RRWheelTmpHighDTC_raw32] -> VDDM_RRWheelTmpHighDTC_raw32/1
  [VDDM_LRWheelTmpHighDTC_raw32] -> VDDM_LRWheelTmpHighDTC_raw32/1
  [VDDM_RFWheelTmpHighDTC_raw32] -> VDDM_RFWheelTmpHighDTC_raw32/1
  [VDDM_LFWheelTmpHighDTC_raw32] -> VDDM_LFWheelTmpHighDTC_raw32/1
  [VDDM_RRPressIndiDTC_raw32] -> VDDM_RRPressIndiDTC_raw32/1
  [VDDM_LRPressIndiDTC_raw32] -> VDDM_LRPressIndiDTC_raw32/1
  [VDDM_RFPressIndiDTC_raw32] -> VDDM_RFPressIndiDTC_raw32/1
  [VDDM_LFPressIndiDTC_raw32] -> VDDM_LFPressIndiDTC_raw32/1
  TPM/12(VDDM_RRWheelTmpHighDTC_raw32) -> [VDDM_RRWheelTmpHighDTC_raw32]
  TPM/11(VDDM_LRWheelTmpHighDTC_raw32) -> [VDDM_LRWheelTmpHighDTC_raw32]
  TPM/10(VDDM_RFWheelTmpHighDTC_raw32) -> [VDDM_RFWheelTmpHighDTC_raw32]
  TPM/9(VDDM_LFWheelTmpHighDTC_raw32) -> [VDDM_LFWheelTmpHighDTC_raw32]
  TPM/8(VDDM_RRPressIndiDTC_raw32) -> [VDDM_RRPressIndiDTC_raw32]
  TPM/7(VDDM_LRPressIndiDTC_raw32) -> [VDDM_LRPressIndiDTC_raw32]
  TPM/6(VDDM_RFPressIndiDTC_raw32) -> [VDDM_RFPressIndiDTC_raw32]
  TPM/5(VDDM_LFPressIndiDTC_raw32) -> [VDDM_LFPressIndiDTC_raw32]
  VTPM_RRPressIndi_enum/1 -> TPM/11(VTPM_RRPressIndi_enum)
  VTPM_LRPressIndi_enum/1 -> TPM/10(VTPM_LRPressIndi_enum)
  VTPM_RFWheelTmpIndi_flg/1 -> TPM/13(VTPM_RFWheelTmpIndi_flg)
  VTPM_LFPressIndi_enum/1 -> TPM/8(VTPM_LFPressIndi_enum)
  VTPM_LFWheelTmpIndi_flg/1 -> TPM/12(VTPM_LFWheelTmpIndi_flg)
  VTPM_RFPressIndi_enum/1 -> TPM/9(VTPM_RFPressIndi_enum)
  VTPM_RRWheelTmpIndi_flg/1 -> TPM/15(VTPM_RRWheelTmpIndi_flg)
  VTPM_LRWheelTmpIndi_flg/1 -> TPM/14(VTPM_LRWheelTmpIndi_flg)
  [VINP_MCUWarnRNidec_enum] -> TQD/33(VINP_MCUWarnRNidec_enum)
  [VINP_MCUWarnFNidec_enum] -> TQD/32(VINP_MCUWarnFNidec_enum)
  [VDDM_RRBatwarnDTC_raw32] -> VDDM_RRBatwarnDTC_raw32/1
  [VDDM_LRBatwarnDTC_raw32] -> VDDM_LRBatwarnDTC_raw32/1
  [VDDM_RFBatwarnDTC_raw32] -> VDDM_RFBatwarnDTC_raw32/1
  [VDDM_LFBatwarnDTC_raw32] -> VDDM_LFBatwarnDTC_raw32/1
  TPM/4(VDDM_RRBatwarnDTC_raw32) -> [VDDM_RRBatwarnDTC_raw32]
  TPM/3(VDDM_LRBatwarnDTC_raw32) -> [VDDM_LRBatwarnDTC_raw32]
  TPM/2(VDDM_RFBatwarnDTC_raw32) -> [VDDM_RFBatwarnDTC_raw32]
  TPM/1(VDDM_LFBatwarnDTC_raw32) -> [VDDM_LFBatwarnDTC_raw32]
  VTPM_RRBatwarn_flg/1 -> TPM/7(VTPM_RRBatwarn_flg)
  VTPM_LRBatwarn_flg/1 -> TPM/6(VTPM_LRBatwarn_flg)
  VTPM_RFBatwarn_flg/1 -> TPM/5(VTPM_RFBatwarn_flg)
  VTPM_LFBatwarn_flg/1 -> TPM/4(VTPM_LFBatwarn_flg)
  [DTC_clear_request] -> TPM/3(DTC_clear_request)
  [VPMM_PowerSta_enum] -> TPM/2(VPMM_PowerSta_enum)
  [task_time_s] -> TPM/1(task_time_s)
  Ground19/1 -> VDDM_ESC7RCErrDTC_raw32/1  "VDDM_ESC7RCErrDTC_raw32"
  [VDDM_MCUF1CSErrDTC_raw32] -> VDDM_MCUF1CSErrDTC_raw32/1
  [VDDM_Shifter1CSErrDTC_raw32] -> VDDM_Shifter1CSErrDTC_raw32/1
  [VDDM_MCUR1RCErrDTC_raw32] -> VDDM_MCUR1RCErrDTC_raw32/1
  [VDDM_ESC1RCErrDTC_raw32] -> VDDM_ESC1RCErrDTC_raw32/1
  Ground20/1 -> VDDM_ESC7CSErrDTC_raw32/1  "VDDM_ESC7CSErrDTC_raw32"
  [VDDM_ESC5RCErrDTC_raw32] -> VDDM_ESC5RCErrDTC_raw32/1
  [VDDM_Shifter1RCErrDTC_raw32] -> VDDM_Shifter1RCErrDTC_raw32/1
  [VDDM_MCUR1CSErrDTC_raw32] -> VDDM_MCUR1CSErrDTC_raw32/1
  [VDDM_RrMCUTqErrDTC_raw32] -> VDDM_RrMCUTqErrDTC_raw32/1
  [VDDM_ESC5CSErrDTC_raw32] -> VDDM_ESC5C  SErrDTC_raw32/1
  [VDDM_FrMCUTqErrDTC_raw32] -> VDDM_FrMCUTqErrDTC_raw32/1
  [VDDM_ESC1CSErrDTC_raw32] -> VDDM_ESC1CSErrDTC_raw32/1
  [VDDM_MCUF1RCErrDTC_raw32] -> VDDM_MCUF1RCErrDTC_raw32/1
  VDDM_ESC1RCErr_flg/1 -> [VDDM_ESC1RCErr_flg]
  VTQR_RrTMTqReq_Nm/1 -> [VTQR_RrTMTqReq_Nm]
  VDDM_ESC5CSErr_flg/1 -> [VDDM_ESC5CSErr_flg]
  VDDM_Shifter1CSErr_flg/1 -> [VDDM_Shifter1CSErr_flg]
  VDDM_MCUNF1RCErr_flg/1 -> [VDDM_MCUNF1RCErr_flg]
  VINP_FrEDUDrtStaNidec_flg/1 -> [VINP_FrEDUDrtStaNidec_flg]
  VDDM_ESC1CSErr_flg/1 -> [VDDM_ESC1CSErr_flg]
  VDDM_MCUNR1CSErr_flg/1 -> [VDDM_MCUNR1CSErr_flg]
  VTQR_FrTMTqReq_Nm/1 -> [VTQR_FrTMTqReq_Nm]
  VDDM_MCUNF1CSErr_flg/1 -> [VDDM_MCUNF1CSErr_flg]
  VINP_RrEDURealTMTqNidec_Nm/1 -> [VINP_RrEDURealTMTqNidec_Nm]
  VDDM_ESC5RCErr_flg/1 -> [VDDM_ESC5RCErr_flg]
  VDDM_Shifter1RCErr_flg/1 -> [VDDM_Shifter1RCErr_flg]
  VDDM_MCUNR1RCErr_flg/1 -> [VDDM_MCUNR1RCErr_flg]
  VINP_FrEDURealTMTqNidec_Nm/1 -> [VINP_FrEDURealTMTqNidec_Nm]
  VINP_RrEDUDrtStaNidec_flg/1 -> [VINP_RrEDUDrtStaNidec_flg]
  [VDDM_ESC5CSErrCFS_flg] -> VMC_DDM/38(VDDM_ESC5CSErrCFS_flg)
  [VDDM_ESC5RCErrCFS_flg] -> VMC_DDM/37(VDDM_ESC5RCErrCFS_flg)
  [VDDM_ESC1CSErrCFS_flg] -> VMC_DDM/35(VDDM_ESC1CSErrCFS_flg)
  [VDDM_ESC1RCErrCFS_flg] -> VMC_DDM/34(VDDM_ESC1RCErrCFS_flg)
  [VDDM_MCUNR1CSErrCFS_flg] -> VMC_DDM/26(VDDM_MCUNR1CSErrCFS_flg)
  [VDDM_MCUNR1RCErrCFS_flg] -> VMC_DDM/25(VDDM_MCUNR1RCErrCFS_flg)
  [VDDM_MCUNF1CSErrCFS_flg] -> VMC_DDM/21(VDDM_MCUNF1CSErrCFS_flg)
  [VDDM_MCUNF1RCErrCFS_flg] -> VMC_DDM/20(VDDM_MCUNF1RCErrCFS_flg)
  TQD/32(VDDM_ESC5CSErrCFS_flg) -> [VDDM_ESC5CSErrCFS_flg]
  TQD/31(VDDM_ESC5RCErrCFS_flg) -> [VDDM_ESC5RCErrCFS_flg]
  TQD/30(VDDM_ESC5NoComCFS_flg) -> [VDDM_ESC5NoComCFS_flg]
  TQD/29(VDDM_ESC1CSErrCFS_flg) -> [VDDM_ESC1CSErrCFS_flg]
  TQD/28(VDDM_ESC1RCErrCFS_flg) -> [VDDM_ESC1RCErrCFS_flg]
  TQD/27(VDDM_ESC1NoComCFS_flg) -> [VDDM_ESC1NoComCFS_flg]
  TQD/26(VDDM_MCUNR1CSErrCFS_flg) -> [VDDM_MCUNR1CSErrCFS_flg]
  TQD/25(VDDM_MCUNR1RCErrCFS_flg) -> [VDDM_MCUNR1RCErrCFS_flg]
  TQD/24(VDDM_MCUNR1NoComCFS_flg) -> [VDDM_MCUNR1NoComCFS_flg]
  TQD/23(VDDM_MCUNF1CSErrCFS_flg) -> [VDDM_MCUNF1CSErrCFS_flg]
  TQD/22(VDDM_MCUNF1RCErrCFS_flg) -> [VDDM_MCUNF1RCErrCFS_flg]
  TQD/21(VDDM_MCUNF1NoComCFS_flg) -> [VDDM_MCUNF1NoComCFS_flg]
  [VDDM_ESC5CSErr_flg] -> TQD/24(VDDM_ESC5CSErr_flg)
  TQD/17(VDDM_ESC5RCErrDTC_raw32) -> [VDDM_ESC5RCErrDTC_raw32]
  TQD/11(VDDM_MCUF1CSErrDTC_raw32) -> [VDDM_MCUF1CSErrDTC_raw32]
  TQD/1(VDDM_APS1SigOoRDTC_raw32) -> [VDDM_APS1SigOoRDTC_raw32]
  [No_CAN1_BUS_OFF] -> TQD/9(No_CAN1_BUS_OFF)
  TQD/13(VDDM_Shifter1RCErrDTC_raw32) -> [VDDM_Shifter1RCErrDTC_raw32]
  [VINP_FrEDUDrtStaNidec_flg] -> TQD/25(VINP_FrEDUDrtStaNidec_flg)
  TQD/16(VDDM_ESC1CSErrDTC_raw32) -> [VDDM_ESC1CSErrDTC_raw32]
  TQD/15(VDDM_ESC1RCErrDTC_raw32) -> [VDDM_ESC1RCErrDTC_raw32]
  [VINP_RrEDUDrtStaNidec_flg] -> TQD/29(VINP_RrEDUDrtStaNidec_flg)
  [VDDM_MCUNR1RCErr_flg] -> TQD/17(VDDM_MCUNR1RCErr_flg)
  [VINP_CANMsgValidMCUNF1_flg] -> TQD/10(VINP_CANMsgValidMCUNF1_flg)
  TQD/9(VDDM_MCUF1RCErrDTC_raw32) -> [VDDM_MCUF1RCErrDTC_raw32]
  [VDDM_ESC1RCErr_flg] -> TQD/21(VDDM_ESC1RCErr_flg)
  TQD/12(VDDM_MCUR1CSErrDTC_raw32) -> [VDDM_MCUR1CSErrDTC_raw32]
  [VDDM_ESC1CSErr_flg] -> TQD/22(VDDM_ESC1CSErr_flg)
  [VINP_RrEDURealTMTqNidec_Nm] -> TQD/30(VINP_RrEDURealTMTqNidec_Nm)
  TQD/18(VDDM_ESC5CSErrDTC_raw32) -> [VDDM_ESC5CSErrDTC_raw32]
  TQD/19(VDDM_FrMCUTqErrDTC_raw32) -> [VDDM_FrMCUTqErrDTC_raw32]
  [task_time_s] -> TQD/6(task_time_s)
  [DTC_clear_request] -> TQD/7(DTC_clear_request)
  [VDDM_Shifter1CSErr_flg] -> TQD/20(VDDM_Shifter1CSErr_flg)
  TQD/14(VDDM_Shifter1CSErrDTC_raw32) -> [VDDM_Shifter1CSErrDTC_raw32]
  [VINP_CANMsgValidShifter1_flg] -> TQD/12(VINP_CANMsgValidShifter1_flg)
  [VDDM_ESC5RCErr_flg] -> TQD/23(VDDM_ESC5RCErr_flg)
  [VTQR_RrTMTqReq_Nm] -> TQD/31(VTQR_RrTMTqReq_Nm)
  [VDHP_EAPS12RangeSta_enum] -> TQD/4(VDHP_EAPS12RangeSta_enum)
  [VDDM_MCUNR1CSErr_flg] -> TQD/18(VDDM_MCUNR1CSErr_flg)
  TQD/8(VDDM_ESC5NoComDTC_raw32) -> [VDDM_ESC5NoComDTC_raw32]
  [VDDM_Shifter1RCErr_flg] -> TQD/19(VDDM_Shifter1RCErr_flg)
  [VINP_CANMsgValidESC5_flg] -> TQD/14(VINP_CANMsgValidESC5_flg)
  TQD/3(VDDM_APSCorrErrDTC_raw32) -> [VDDM_APSCorrErrDTC_raw32]
  TQD/6(VDDM_Shifter1NoComDTC_raw32) -> [VDDM_Shifter1NoComDTC_raw32]
  TQD/4(VDDM_MCUF1NoComDTC_raw32) -> [VDDM_MCUF1NoComDTC_raw32]
  [VDDM_MCUNF1RCErr_flg] -> TQD/15(VDDM_MCUNF1RCErr_flg)
  [VINP_CANMsgValidMCUNR1_flg] -> TQD/11(VINP_CANMsgValidMCUNR1_flg)
  TQD/7(VDDM_ESC1NoComDTC_raw32) -> [VDDM_ESC1NoComDTC_raw32]
  [VDHP_EAPCRBAD_flg] -> TQD/5(VDHP_EAPCRBAD_flg)
  [VTQR_FrTMTqReq_Nm] -> TQD/28(VTQR_FrTMTqReq_Nm)
  [VINP_VehSpeed_kph] -> TQD/26(VINP_VehSpeed_kph)
  TQD/10(VDDM_MCUR1RCErrDTC_raw32) -> [VDDM_MCUR1RCErrDTC_raw32]
  [No_CAN3_BUS_OFF] -> TQD/8(No_CAN3_BUS_OFF)
  [VINP_CANMsgValidESC1_flg] -> TQD/13(VINP_CANMsgValidESC1_flg)
  [VDDM_MCUNF1CSErr_flg] -> TQD/16(VDDM_MCUNF1CSErr_flg)
  [VPMM_PwrStaSW_enum] -> TQD/1(VPMM_SysPwrSta_enum)
  TQD/2(VDDM_APS2SigOoRDTC_raw32) -> [VDDM_APS2SigOoRDTC_raw32]
  TQD/5(VDDM_MCUR1NoComDTC_raw32) -> [VDDM_MCUR1NoComDTC_raw32]
  TQD/20(VDDM_RrMCUTqErrDTC_raw32) -> [VDDM_RrMCUTqErrDTC_raw32]
  [VINP_FrEDURealTMTqNidec_Nm] -> TQD/27(VINP_FrEDURealTMTqNidec_Nm)
  [VINP_VehSpeed_kph] -> VMC_DDM/18(VINP_VehSpeed_kph)
  [VDDM_CCUSigErrDetDTC_raw32] -> VDDM_CCUSigErrDetDTC_raw32/1
  Ground13/1 -> VDDM_FCM5CSErrDTC_raw32/1  "VDDM_FCM5CSErrDTC_raw32"
  Ground12/1 -> VDDM_FCM5NoComDTC_raw32/1  "VDDM_FCM5NoComDTC_raw32"
  [VDDM_RrMCUSigErrDetDTC_raw32] -> VDDM_RrMCUSigErrDetDTC_raw32/1
  [VDDM_ACCAccelCmdErrDetDTC_raw32] -> VDDM_ACCAccelCmdErrDetDTC_raw32/1
  [VDDM_BMSSigErrDetDTC_raw32] -> VDDM_BMSSigErrDetDTC_raw32/1
  Ground10/1 -> VDDM_FCM4NoComDTC_raw32/1  "VDDM_FCM4NoComDTC_raw32"
  Ground15/1 -> VDDM_ACCMalfuncDetDTC_raw32/1  "VDDM_ACCMalfuncDetDTC_raw32"
  Ground16/1 -> VDDM_CCMalfuncDetDTC_raw32/1  "VDDM_CCMalfuncDetDTC_raw32"
  Ground17/1 -> VDDM_MSAMalfuncDetDTC_raw32/1  "VDDM_MSAMalfuncDetDTC_raw32"
  Ground14/1 -> VDDM_ZoneSCPNoComDTC_raw32/1  "VDDM_ZoneSCPNoComDTC_raw32"
  [VDDM_FrMCUSigErrDetDTC_raw32] -> VDDM_FrMCUSigErrDetDTC_raw32/1
  Ground11/1 -> VDDM_FCM4CSErrDTC_raw32/1  "VDDM_FCM4CSErrDTC_raw32"
  [VDDM_FCMACCSigErrDetDTC_raw32] -> VDDM_FCMACCSigErrDetDTC_raw32/1
  Ground18/1 -> VDDM_ISAMalfuncDetDTC_raw32/1  "VDDM_ISAMalfuncDetDTC_raw32"
  Ground9/1 -> VDDM_FCM3CSErrDTC_raw32/1  "VDDM_FCM3CSErrDTC_raw32"
  Ground8/1 -> VDDM_FCM3RCErrDTC_raw32/1  "VDDM_FCM3RCErrDTC_raw32"
  Ground7/1 -> VDDM_FCM3NoComDTC_raw32/1  "VDDM_FCM3NoComDTC_raw32"
  Ground6/1 -> VDDM_FCM2CSErrDTC_raw32/1  "VDDM_FCM2CSErrDTC_raw32"
  Ground5/1 -> VDDM_FCM2RCErrDTC_raw32/1  "VDDM_FCM2RCErrDTC_raw32"
  Ground2/1 -> VDDM_FCM2NoComDTC_raw32/1  "VDDM_FCM2NoComDTC_raw32"
  [VDDM_ESC5NoComCFS_flg] -> VMC_DDM/36(VDDM_ESC5NoComCFS_flg)
  [VDDM_ESC1NoComCFS_flg] -> VMC_DDM/33(VDDM_ESC1NoComCFS_flg)
  [VDDM_MCUNR1NoComCFS_flg] -> VMC_DDM/24(VDDM_MCUNR1NoComCFS_flg)
  [VDDM_MCUNF1NoComCFS_flg] -> VMC_DDM/19(VDDM_MCUNF1NoComCFS_flg)
  [VDDM_C3CCU2CSCFS_flg] -> VMC_DDM/29(VDDM_C3CCU2CSCFS_flg)
  [VDDM_C3CCU2RCCFS_flg] -> VMC_DDM/28(VDDM_C3CCU2RCCFS_flg)
  [VDDM_C3CCU2LCCFS_flg] -> VMC_DDM/27(VDDM_C3CCU2LCCFS_flg)
  [VDDM_C3BMS6CSCFS_flg] -> VMC_DDM/11(VDDM_C3BMS6CSCFS_flg)
  [VDDM_C3BMS6RCCFS_flg] -> VMC_DDM/10(VDDM_C3BMS6RCCFS_flg)
  [VDDM_C3BMS6LCCFS_flg] -> VMC_DDM/9(VDDM_C3BMS6LCCFS_flg)
  [VINP_DCDCFaultSta_enum] -> VMC_DDM/30(VINP_DCDCFaultSta_enum)
  [VINP_DCDCFaultSta_enum] -> PMM/18(VINP_DCDCFaultSta_enum)
  [VINP_MCUWarnRNidec_enum] -> VMC_DDM/23(VINP_MCUWarnRNidec_enum)
  [VINP_MCUWarnFNidec_enum] -> VMC_DDM/22(VINP_MCUWarnFNidec_enum)
  [VINP_MCUWarnRNidec_enum] -> PMM/21(VINP_MCUWarnRNidec_enum)
  [VINP_MCUWarnFNidec_enum] -> PMM/20(VINP_MCUWarnFNidec_enum)
  [VINP_BMSWarn8_flg] -> VMC_DDM/12(VINP_BMSWarn8_flg)
  [VINP_BMSWarn7_flg] -> VMC_DDM/13(VINP_BMSWarn7_flg)
  [VINP_BMSWarn6_flg] -> VMC_DDM/14(VINP_BMSWarn6_flg)
  [VINP_BMSWarn5_flg] -> VMC_DDM/15(VINP_BMSWarn5_flg)
  [VINP_BMSWarn4_flg] -> VMC_DDM/16(VINP_BMSWarn4_flg)
  [VINP_BMSWarn4_flg] -> PMM/13(VINP_BMSWarn4_flg)
  VINP_BMSWarn4_flg/1 -> [VINP_BMSWarn4_flg]
  [VINP_BMSWarn8_flg] -> PMM/17(VINP_BMSWarn8_flg)
  [VINP_BMSWarn7_flg] -> PMM/16(VINP_BMSWarn7_flg)
  [VINP_BMSWarn6_flg] -> PMM/15(VINP_BMSWarn6_flg)
  [VINP_BMSWarn5_flg] -> PMM/14(VINP_BMSWarn5_flg)
  VINP_BMSWarn8_flg/1 -> [VINP_BMSWarn8_flg]
  VINP_BMSWarn7_flg/1 -> [VINP_BMSWarn7_flg]
  VINP_BMSWarn6_flg/1 -> [VINP_BMSWarn6_flg]
  VINP_BMSWarn5_flg/1 -> [VINP_BMSWarn5_flg]
  [No_CAN3_BUS_OFF] -> VMC_DDM/41(No_CAN3_BUS_OFF)
  [No_CAN1_BUS_OFF] -> VMC_DDM/40(No_CAN1_BUS_OFF)
  [VPMM_PowerSta_enum] -> VMC_DDM/6(VPMM_PowerSta_enum)
  [DTC_clear_request] -> VMC_DDM/8(DTC_clear_request)
  [task_time_s] -> VMC_DDM/1(task_time_s)
  [VDDM_FCLUSSDTC_raw32] -> VDDM_FCLUSSDTC_raw32/1
  [VDDM_RLLUSSDTC_raw32] -> VDDM_RLLUSSDTC_raw32/1
  [VDDM_RMLUSSDTC_raw32] -> VDDM_RMLUSSDTC_raw32/1
  [VDDM_FMLUSSDTC_raw32] -> VDDM_FMLUSSDTC_raw32/1
  [VDDM_RCLUSSDTC_raw32] -> VDDM_RCLUSSDTC_raw32/1
  [VDDM_RMRUSSDTC_raw32] -> VDDM_RMRUSSDTC_raw32/1
  [VDDM_RCRUSSDTC_raw32] -> VDDM_RCRUSSDTC_raw32/1
  [VDDM_FMRUSSDTC_raw32] -> VDDM_FMRUSSDTC_raw32/1
  [VDDM_RLRUSSDTC_raw32] -> VDDM_RLRUSSDTC_raw32/1
  [VDDM_FCRUSSDTC_raw32] -> VDDM_FCRUSSDTC_raw32/1
  [VDDM_FLRUSSDTC_raw32] -> VDDM_FLRUSSDTC_raw32/1
  [VDDM_FLLUSSDTC_raw32] -> VDDM_FLLUSSDTC_raw32/1
  [VPMM_PwrStaSW_enum] -> APM/14(VPMM_SysPwrSta_enum)
  VAPM_USSStaFLL_flg/1 -> APM/9(VAPM_USSStaFLL_flg)
  APM/1(VDDM_FCLUSSDTC_raw32) -> [VDDM_FCLUSSDTC_raw32]
  APM/11(VDDM_RLLUSSDTC_raw32) -> [VDDM_RLLUSSDTC_raw32]
  APM/5(VDDM_RCLUSSDTC_raw32) -> [VDDM_RCLUSSDTC_raw32]
  VAPM_USSStaRMR_flg/1 -> APM/7(VAPM_USSStaRMR_flg)
  APM/6(VDDM_RMLUSSDTC_raw32) -> [VDDM_RMLUSSDTC_raw32]
  VAPM_USSStaRLR_flg/1 -> APM/12(VAPM_USSStaRLR_flg)
  APM/4(VDDM_FCRUSSDTC_raw32) -> [VDDM_FCRUSSDTC_raw32]
  APM/9(VDDM_FLLUSSDTC_raw32) -> [VDDM_FLLUSSDTC_raw32]
  APM/7(VDDM_RMRUSSDTC_raw32) -> [VDDM_RMRUSSDTC_raw32]
  VAPM_USSStaFMR_flg/1 -> APM/3(VAPM_USSStaFMR_flg)
  VAPM_USSStaFLR_flg/1 -> APM/10(VAPM_USSStaFLR_flg)
  APM/8(VDDM_RCRUSSDTC_raw32) -> [VDDM_RCRUSSDTC_raw32]
  VAPM_USSStaRLL_flg/1 -> APM/11(VAPM_USSStaRLL_flg)
  VAPM_USSStaRCR_flg/1 -> APM/8(VAPM_USSStaRCR_flg)
  VAPM_USSStaRCL_flg/1 -> APM/5(VAPM_USSStaRCL_flg)
  APM/10(VDDM_FLRUSSDTC_raw32) -> [VDDM_FLRUSSDTC_raw32]
  VAPM_USSStaFCR_flg/1 -> APM/4(VAPM_USSStaFCR_flg)
  VAPM_USSStaRML_flg/1 -> APM/6(VAPM_USSStaRML_flg)
  APM/12(VDDM_RLRUSSDTC_raw32) -> [VDDM_RLRUSSDTC_raw32]
  VAPM_USSStaFCL_flg/1 -> APM/1(VAPM_USSStaFCL_flg)
  VAPM_USSStaFML_flg/1 -> APM/2(VAPM_USSStaFML_flg)
  APM/3(VDDM_FMRUSSDTC_raw32) -> [VDDM_FMRUSSDTC_raw32]
  APM/2(VDDM_FMLUSSDTC_raw32) -> [VDDM_FMLUSSDTC_raw32]
  [DTC_clear_request] -> APM/13(DTC_clear_request)
  Data Type Conversion56/1 -> [DTC_clear_request]
  [DTC_clear_request] -> BCM/6(DTC_clear_request)
  [VDDM_ESC1NoComCFS_flg] -> Chart/29(VDDM_ESC1NoComCFS_flg)
  [VDDM_ESC5NoComCFS_flg] -> Chart/32(VDDM_ESC5NoComCFS_flg)
  [VDDM_MCUNF1NoComCFS_flg] -> Chart/52(VDDM_MCUNF1NoComCFS_flg)
  [VDDM_MCUNR1NoComCFS_flg] -> Chart/55(VDDM_MCUNR1NoComCFS_flg)
  [VDDM_Shifter1NoComCFS_flg] -> Chart/63(VDDM_Shifter1NoComCFS_flg)
  VINP_CANMsgValidMCUNR1_flg/1 -> [VINP_CANMsgValidMCUNR1_flg]
  VINP_CANMsgValidMCUNF1_flg/1 -> [VINP_CANMsgValidMCUNF1_flg]
  VINP_CANMsgValidESC1_flg/1 -> [VINP_CANMsgValidESC1_flg]
  VINP_CANMsgValidESC5_flg/1 -> [VINP_CANMsgValidESC5_flg]
  [VDDM_Shifter1NoComDTC_raw32] -> VDDM_Shifter1NoComDTC_raw32/1
  VINP_CANMsgValidShifter1_flg/1 -> [VINP_CANMsgValidShifter1_flg]
  Ground/1 -> VDDM_ESC7NoComDTC_raw32/1  "VDDM_ESC7NoComDTC_raw32"
  [VDDM_ESC5NoComDTC_raw32] -> VDDM_ESC5NoComDTC_raw32/1
  [VDDM_ESC1NoComDTC_raw32] -> VDDM_ESC1NoComDTC_raw32/1
  [VDDM_MCUR1NoComDTC_raw32] -> VDDM_MCUR1NoComDTC_raw32/1
  [VDDM_MCUF1NoComDTC_raw32] -> VDDM_MCUF1NoComDTC_raw32/1
  Constant1/1 -> Switch/3
  Constant15/1 -> Switch/2
  [VDDM_DiagFLTSDTC_raw32] -> VDDM_DiagFLTSDTC_raw32/1
  [VDDM_DiagFRTSDTC_raw32] -> VDDM_DiagFRTSDTC_raw32/1
  [VDDM_DiagRLTSDTC_raw32] -> VDDM_DiagRLTSDTC_raw32/1
  [VDDM_DiagHCrashDTC_raw32] -> VDDM_DiagHCrashDTC_raw32/1
  [VDDM_DiagRRTSDTC_raw32] -> VDDM_DiagRRTSDTC_raw32/1
  BCM/5(VDDM_DiagRRTSDTC_raw32) -> [VDDM_DiagRRTSDTC_raw32]
  BCM/4(VDDM_DiagRLTSDTC_raw32) -> [VDDM_DiagRLTSDTC_raw32]
  BCM/3(VDDM_DiagFRTSDTC_raw32) -> [VDDM_DiagFRTSDTC_raw32]
  BCM/2(VDDM_DiagFLTSDTC_raw32) -> [VDDM_DiagFLTSDTC_raw32]
  VBCM_DiagRRTS_flg/1 -> BCM/5(VBCM_DiagRRTS_flg)
  VBCM_DiagRLTS_flg/1 -> BCM/4(VBCM_DiagRLTS_flg)
  VBCM_DiagFRTS_flg/1 -> BCM/3(VBCM_DiagFRTS_flg)
  VBCM_DiagFLTS_flg/1 -> BCM/2(VBCM_DiagFLTS_flg)
  BCM/1(VDDM_DiagHCrashDTC_raw32) -> [VDDM_DiagHCrashDTC_raw32]
  VBCM_DiagHCrash_flg/1 -> BCM/1(VBCM_DiagHCrash_flg)
  DTC_clear_request/1 -> Data Type Conversion56/1
  Data Type Conversion49/1 -> Equal/1
  [VPMM_PwrStaSW_enum] -> Data Type Conversion49/1
  Latch/1 -> Detect Increase/1
  Detect Increase/1 -> VDDM_EnterNewOperCyc_flg/1  "VDDM_EnterNewOperCyc_flg"
  Equal/1 -> Latch/1
  Constant/1 -> Equal/2
  [VDDM_APSCorrErrDTC_raw32] -> VDDM_APSCorrErrDTC_raw32/1
  [VDDM_APS2SigOoRDTC_raw32] -> VDDM_APS2SigOoRDTC_raw32/1
  [VDDM_APS1SigOoRDTC_raw32] -> VDDM_APS1SigOoRDTC_raw32/1
  [VDDM_APSCorrErrCFS_flg] -> Chart/71(VDDM_APSCorrErrCFS_flg)
  [VDDM_APS2SigOoRCFS_flg] -> Chart/70(VDDM_APS2SigOoRCFS_flg)
  [VDDM_APS1SigOoRCFS_flg] -> Chart/69(VDDM_APS1SigOoRCFS_flg)
  VDHP_EAPCRBAD_flg/1 -> [VDHP_EAPCRBAD_flg]
  Chart/3(VDDM_limphome_enum) -> Terminator1/1  "VDDM_limphome_enum"
  Chart/2(VDDM_EmergencyPwrDown_flg) -> Terminator/1  "VDDM_EmergencyPwrDown_flg"
  Data Type Conversion1/1 -> VDDM_VehMalfunLevel_enum/1  "VDDM_VehMalfunLevel_enum"
  [VDDM_ESC5CSErrCFS_flg] -> PMM/68(VDDM_ESC5CSErrCFS_flg)
  [VDDM_ESC5RCErrCFS_flg] -> PMM/67(VDDM_ESC5RCErrCFS_flg)
  [VDDM_ESC5NoComCFS_flg] -> PMM/66(VDDM_ESC5NoComCFS_flg)
  [VDDM_MCUNR1NoComCFS_flg] -> PMM/65(VDDM_MCUNR1NoComCFS_flg)
  [VDDM_MCUNF1NoComCFS_flg] -> PMM/64(VDDM_MCUNF1NoComCFS_flg)
  [ZoneFrMalfunLevel_enum] -> Chart/68(ZoneFrMalfunLevel_enum)
  [VINP_ZoneDrMalfunLevel_enum] -> Chart/67(ZoneDrMalfunLevel_enum)
  [VDDM_Shifter1RCErrCFS_flg] -> Chart/64(VDDM_Shifter1RCErrCFS_flg)
  [VDDM_Shifter1CSErrCFS_flg] -> Chart/62(VDDM_Shifter1CSErrCFS_flg)
  [VDDM_MCUNR1RCErrCFS_flg] -> Chart/56(VDDM_MCUNR1RCErrCFS_flg)
  [VDDM_MCUNR1CSErrCFS_flg] -> Chart/54(VDDM_MCUNR1CSErrCFS_flg)
  [VDDM_MCUNF1RCErrCFS_flg] -> Chart/53(VDDM_MCUNF1RCErrCFS_flg)
  [VDDM_MCUNF1CSErrCFS_flg] -> Chart/51(VDDM_MCUNF1CSErrCFS_flg)
  [VDDM_ESC5RCErrCFS_flg] -> Chart/33(VDDM_ESC5RCErrCFS_flg)
  [VDDM_ESC5CSErrCFS_flg] -> Chart/31(VDDM_ESC5CSErrCFS_flg)
  [VDDM_ESC1RCErrCFS_flg] -> Chart/30(VDDM_ESC1RCErrCFS_flg)
  [VDDM_ESC1CSErrCFS_flg] -> Chart/28(VDDM_ESC1CSErrCFS_flg)
  [VDDM_TailgaSWCFS_flg] -> Chart/66(VDDM_TailgaSWCFS_flg)
  [VDDM_HoodSWCFS_flg] -> Chart/65(VDDM_HoodSWCFS_flg)
  [VDDM_RRDoorSWCFS_flg] -> Chart/61(VDDM_RRDoorSWCFS_flg)
  [VDDM_RLDoorSWCFS_flg] -> Chart/60(VDDM_RLDoorSWCFS_flg)
  [VDDM_ONtoRdyCFS_flg] -> Chart/59(VDDM_ONtoRdyCFS_flg)
  [VDDM_OBC4PreCFS_flg] -> Chart/58(VDDM_OBC4PreCFS_flg)
  [VDDM_MidLvSaChkCFS_flg] -> Chart/57(VDDM_MidLvSaChkCFS_flg)
  [VDDM_MCUDisCFS_flg] -> Chart/50(VDDM_MCUDisCFS_flg)
  [VDDM_MCUActCFS_flg] -> Chart/49(VDDM_MCUActCFS_flg)
  [VDDM_MCU4PreCFS_flg] -> Chart/48(VDDM_MCU4PreCFS_flg)
  [VDDM_Lv4ErrCFS_flg] -> Chart/1(VDDM_Lv4ErrCFS_flg)
  [VDDM_Lv3ErrCFS_flg] -> Chart/47(VDDM_Lv3ErrCFS_flg)
  [VDDM_Lv2ErrCFS_flg] -> Chart/46(VDDM_Lv2ErrCFS_flg)
  [VDDM_Lv1ErrCFS_flg] -> Chart/45(VDDM_Lv1ErrCFS_flg)
  [VDDM_LVSupLoCFS_flg] -> Chart/44(VDDM_LVSupLoCFS_flg)
  [VDDM_LVSupHiCFS_flg] -> Chart/43(VDDM_LVSupHiCFS_flg)
  [VDDM_KeyAuthCFS_flg] -> Chart/41(VDDM_KeyAuthCFS_flg)
  [VDDM_IniLVLoCFS_flg] -> Chart/40(VDDM_IniLVLoCFS_flg)
  [VDDM_HiLvSaChkCFS_flg] -> Chart/39(VDDM_HiLvSaChkCFS_flg)
  [VDDM_HVRlyOpCFS_flg] -> Chart/38(VDDM_HVRlyOpCFS_flg)
  [VDDM_HVRlyCloCFS_flg] -> Chart/37(VDDM_HVRlyCloCFS_flg)
  [VDDM_HVB4PreCFS_flg] -> Chart/36(VDDM_HVB4PreCFS_flg)
  [VDDM_FRDoorSWCFS_flg] -> Chart/35(VDDM_FRDoorSWCFS_flg)
  [VDDM_FLDoorSWCFS_flg] -> Chart/34(VDDM_FLDoorSWCFS_flg)
  [VDDM_DrStSWCFS_flg] -> Chart/25(VDDM_DrStSWCFS_flg)
  [VDDM_DCDCEnaCFS_flg] -> Chart/24(VDDM_DCDCEnaCFS_flg)
  [VDDM_DCDCDisCFS_flg] -> Chart/23(VDDM_DCDCDisCFS_flg)
  [VDDM_DCDC4PreCFS_flg] -> Chart/22(VDDM_DCDC4PreCFS_flg)
  [VDDM_C3CCU2RCCFS_flg] -> Chart/21(VDDM_C3CCU2RCCFS_flg)
  [VDDM_C3CCU2LCCFS_flg] -> Chart/20(VDDM_C3CCU2LCCFS_flg)
  [VDDM_C3CCU2CSCFS_flg] -> Chart/19(VDDM_C3CCU2CSCFS_flg)
  [VDDM_C3CCU1RCCFS_flg] -> Chart/18(VDDM_C3CCU1RCCFS_flg)
  [VDDM_C3CCU1LCCFS_flg] -> Chart/17(VDDM_C3CCU1LCCFS_flg)
  [VDDM_C3CCU1CSCFS_flg] -> Chart/16(VDDM_C3CCU1CSCFS_flg)
  [VDDM_C3BMS6RCCFS_flg] -> Chart/15(VDDM_C3BMS6RCCFS_flg)
  [VDDM_C3BMS6LCCFS_flg] -> Chart/14(VDDM_C3BMS6LCCFS_flg)
  [VDDM_C3BMS6CSCFS_flg] -> Chart/13(VDDM_C3BMS6CSCFS_flg)
  [VDDM_C3BMS1RCCFS_flg] -> Chart/12(VDDM_C3BMS1RCCFS_flg)
  [VDDM_C3BMS1LCCFS_flg] -> Chart/11(VDDM_C3BMS1LCCFS_flg)
  [VDDM_C3BMS1CSCFS_flg] -> Chart/10(VDDM_C3BMS1CSCFS_flg)
  [VDDM_C1ABM1RCCFS_flg] -> Chart/9(VDDM_C1ABM1RCCFS_flg)
  [VDDM_C1ABM1LCCFS_flg] -> Chart/8(VDDM_C1ABM1LCCFS_flg)
  [VDDM_C1ABM1CSCFS_flg] -> Chart/7(VDDM_C1ABM1CSCFS_flg)
  [VDDM_BrkSWNoBacCFS_flg] -> Chart/6(VDDM_BrkSWNoBacCFS_flg)
  [VDDM_BrkSWErrCFS_flg] -> Chart/5(VDDM_BrkSWErrCFS_flg)
  [VDDM_BMSRdyCFS_flg] -> Chart/4(VDDM_BMSRdyCFS_flg)
  [VDDM_5vAPS2OoRCFS_flg] -> Chart/3(VDDM_5vAPS2OoRCFS_flg)
  [VDDM_5vAPS1OoRCFS_flg] -> Chart/2(VDDM_5vAPS1OoRCFS_flg)
  [VDDM_TailgaSWDTC_raw32] -> VDDM_TailgaSWDTC_raw32/1
  [VDDM_HoodSWDTC_raw32] -> VDDM_HoodSWDTC_raw32/1
  [VDDM_RRDoorSWDTC_raw32] -> VDDM_RRDoorSWDTC_raw32/1
  [VDDM_FRDoorSWDTC_raw32] -> VDDM_FRDoorSWDTC_raw32/1
  [VDDM_RLDoorSWDTC_raw32] -> VDDM_RLDoorSWDTC_raw32/1
  [VDDM_FLDoorSWDTC_raw32] -> VDDM_FLDoorSWDTC_raw32/1
  [VDDM_DrStSWDTC_raw32] -> VDDM_DrStSWDTC_raw32/1
  [VDDM_LVSupHiDTC_raw32] -> VDDM_LVSupHiDTC_raw32/1
  [VDDM_LVSupLoDTC_raw32] -> VDDM_LVSupLoDTC_raw32/1
  [VDDM_IniLVLoDTC_raw32] -> VDDM_IniLVLoDTC_raw32/1
  [VDDM_OBC4PreDTC_raw32] -> VDDM_OBC4PreDTC_raw32/1
  [VDDM_MCUActDTC_raw32] -> VDDM_MCUActDTC_raw32/1
  [VDDM_HVRlyOpDTC_raw32] -> VDDM_HVRlyOpDTC_raw32/1
  [VDDM_DCDCDisDTC_raw32] -> VDDM_DCDCDisDTC_raw32/1
  [VDDM_MCUDisDTC_raw32] -> VDDM_MCUDisDTC_raw32/1
  [VDDM_MidLvSaChkDTC_raw32] -> VDDM_MidLvSaChkDTC_raw32/1
  [VDDM_HiLvSaChkDTC_raw32] -> VDDM_HiLvSaChkDTC_raw32/1
  [VDDM_DCDCEnaDTC_raw32] -> VDDM_DCDCEnaDTC_raw32/1
  [VDDM_BMSRdyDTC_raw32] -> VDDM_BMSRdyDTC_raw32/1
  [VDDM_HVRlyCloDTC_raw32] -> VDDM_HVRlyCloDTC_raw32/1
  [VDDM_DCDC4PreDTC_raw32] -> VDDM_DCDC4PreDTC_raw32/1
  [VDDM_MCU4PreDTC_raw32] -> VDDM_MCU4PreDTC_raw32/1
  [VDDM_HVB4PreDTC_raw32] -> VDDM_HVB4PreDTC_raw32/1
  [VDDM_ONtoRdyDTC_raw32] -> VDDM_ONtoRdyDTC_raw32/1
  [VDDM_KeyAuthDTC_raw32] -> VDDM_KeyAuthDTC_raw32/1
  [VDDM_BrkSWNoBacDTC_raw32] -> VDDM_BrkSWNoBacDTC_raw32/1
  [VDDM_BrkSWErrDTC_raw32] -> VDDM_BrkSWErrDTC_raw32/1
  [VDDM_Lv4ErrDTC_raw32] -> VDDM_Lv4ErrDTC_raw32/1
  [VDDM_Lv3ErrDTC_raw32] -> VDDM_Lv3ErrDTC_raw32/1
  [VDDM_Lv2ErrDTC_raw32] -> VDDM_Lv2ErrDTC_raw32/1
  [VDDM_Lv1ErrDTC_raw32] -> VDDM_Lv1ErrDTC_raw32/1
  [VDDM_C1ABM1LCDTC_raw32] -> VDDM_C1ABM1LCDTC_raw32/1
  [VDDM_C1ABM1CSDTC_raw32] -> VDDM_C1ABM1CSDTC_raw32/1
  [VDDM_C1ABM1RCDTC_raw32] -> VDDM_C1ABM1RCDTC_raw32/1
  [VDDM_C3CCU2LCDTC_raw32] -> VDDM_C3CCU2LCDTC_raw32/1
  [VDDM_C3CCU2CSDTC_raw32] -> VDDM_C3CCU2CSDTC_raw32/1
  [VDDM_C3CCU2RCDTC_raw32] -> VDDM_C3CCU2RCDTC_raw32/1
  [VDDM_C3CCU1LCDTC_raw32] -> VDDM_C3CCU1LCDTC_raw32/1
  [VDDM_C3CCU1CSDTC_raw32] -> VDDM_C3CCU1CSDTC_raw32/1
  [VDDM_C3CCU1RCDTC_raw32] -> VDDM_C3CCU1RCDTC_raw32/1
  [VDDM_C3BMS1LCDTC_raw32] -> VDDM_C3BMS1LCDTC_raw32/1
  [VDDM_C3BMS1CSDTC_raw32] -> VDDM_C3BMS1CSDTC_raw32/1
  [VDDM_C3BMS1RCDTC_raw32] -> VDDM_C3BMS1RCDTC_raw32/1
  [VDDM_C3BMS6LCDTC_raw32] -> VDDM_C3BMS6LCDTC_raw32/1
  [VDDM_C3BMS6CSDTC_raw32] -> VDDM_C3BMS6CSDTC_raw32/1
  [VDDM_C3BMS6RCDTC_raw32] -> VDDM_C3BMS6RCDTC_raw32/1
  PMM/47(VDDM_TailgaSWDTC_raw32) -> [VDDM_TailgaSWDTC_raw32]
  PMM/46(VDDM_HoodSWDTC_raw32) -> [VDDM_HoodSWDTC_raw32]
  PMM/45(VDDM_RRDoorSWDTC_raw32) -> [VDDM_RRDoorSWDTC_raw32]
  PMM/44(VDDM_FRDoorSWDTC_raw32) -> [VDDM_FRDoorSWDTC_raw32]
  PMM/43(VDDM_RLDoorSWDTC_raw32) -> [VDDM_RLDoorSWDTC_raw32]
  PMM/42(VDDM_FLDoorSWDTC_raw32) -> [VDDM_FLDoorSWDTC_raw32]
  PMM/41(VDDM_DrStSWDTC_raw32) -> [VDDM_DrStSWDTC_raw32]
  PMM/39(VDDM_LVSupHiDTC_raw32) -> [VDDM_LVSupHiDTC_raw32]
  PMM/38(VDDM_LVSupLoDTC_raw32) -> [VDDM_LVSupLoDTC_raw32]
  PMM/37(VDDM_IniLVLoDTC_raw32) -> [VDDM_IniLVLoDTC_raw32]
  PMM/36(VDDM_OBC4PreDTC_raw32) -> [VDDM_OBC4PreDTC_raw32]
  PMM/35(VDDM_MCUActDTC_raw32) -> [VDDM_MCUActDTC_raw32]
  PMM/34(VDDM_HVRlyOpDTC_raw32) -> [VDDM_HVRlyOpDTC_raw32]
  PMM/33(VDDM_DCDCDisDTC_raw32) -> [VDDM_DCDCDisDTC_raw32]
  PMM/32(VDDM_MCUDisDTC_raw32) -> [VDDM_MCUDisDTC_raw32]
  PMM/31(VDDM_MidLvSaChkDTC_raw32) -> [VDDM_MidLvSaChkDTC_raw32]
  PMM/30(VDDM_HiLvSaChkDTC_raw32) -> [VDDM_HiLvSaChkDTC_raw32]
  PMM/29(VDDM_DCDCEnaDTC_raw32) -> [VDDM_DCDCEnaDTC_raw32]
  PMM/28(VDDM_BMSRdyDTC_raw32) -> [VDDM_BMSRdyDTC_raw32]
  PMM/27(VDDM_HVRlyCloDTC_raw32) -> [VDDM_HVRlyCloDTC_raw32]
  PMM/26(VDDM_DCDC4PreDTC_raw32) -> [VDDM_DCDC4PreDTC_raw32]
  PMM/25(VDDM_MCU4PreDTC_raw32) -> [VDDM_MCU4PreDTC_raw32]
  PMM/24(VDDM_HVB4PreDTC_raw32) -> [VDDM_HVB4PreDTC_raw32]
  PMM/23(VDDM_ONtoRdyDTC_raw32) -> [VDDM_ONtoRdyDTC_raw32]
  PMM/22(VDDM_KeyAuthDTC_raw32) -> [VDDM_KeyAuthDTC_raw32]
  PMM/21(VDDM_BrkSWNoBacDTC_raw32) -> [VDDM_BrkSWNoBacDTC_raw32]
  PMM/20(VDDM_BrkSWErrDTC_raw32) -> [VDDM_BrkSWErrDTC_raw32]
  PMM/19(VDDM_Lv4ErrDTC_raw32) -> [VDDM_Lv4ErrDTC_raw32]
  PMM/18(VDDM_Lv3ErrDTC_raw32) -> [VDDM_Lv3ErrDTC_raw32]
  PMM/17(VDDM_Lv2ErrDTC_raw32) -> [VDDM_Lv2ErrDTC_raw32]
  PMM/16(VDDM_Lv1ErrDTC_raw32) -> [VDDM_Lv1ErrDTC_raw32]
  PMM/15(VDDM_C1ABM1LCDTC_raw32) -> [VDDM_C1ABM1LCDTC_raw32]
  PMM/14(VDDM_C1ABM1CSDTC_raw32) -> [VDDM_C1ABM1CSDTC_raw32]
  PMM/13(VDDM_C1ABM1RCDTC_raw32) -> [VDDM_C1ABM1RCDTC_raw32]
  PMM/12(VDDM_C3CCU2LCDTC_raw32) -> [VDDM_C3CCU2LCDTC_raw32]
  PMM/11(VDDM_C3CCU2CSDTC_raw32) -> [VDDM_C3CCU2CSDTC_raw32]
  PMM/10(VDDM_C3CCU2RCDTC_raw32) -> [VDDM_C3CCU2RCDTC_raw32]
  PMM/9(VDDM_C3CCU1LCDTC_raw32) -> [VDDM_C3CCU1LCDTC_raw32]
  PMM/8(VDDM_C3CCU1CSDTC_raw32) -> [VDDM_C3CCU1CSDTC_raw32]
  PMM/7(VDDM_C3CCU1RCDTC_raw32) -> [VDDM_C3CCU1RCDTC_raw32]
  PMM/6(VDDM_C3BMS1LCDTC_raw32) -> [VDDM_C3BMS1LCDTC_raw32]
  PMM/5(VDDM_C3BMS1CSDTC_raw32) -> [VDDM_C3BMS1CSDTC_raw32]
  PMM/4(VDDM_C3BMS1RCDTC_raw32) -> [VDDM_C3BMS1RCDTC_raw32]
  PMM/3(VDDM_C3BMS6LCDTC_raw32) -> [VDDM_C3BMS6LCDTC_raw32]
  PMM/2(VDDM_C3BMS6CSDTC_raw32) -> [VDDM_C3BMS6CSDTC_raw32]
  PMM/1(VDDM_C3BMS6RCDTC_raw32) -> [VDDM_C3BMS6RCDTC_raw32]
  [No_CAN1_BUS_OFF] -> PMM/61(No_CAN1_BUS_OFF)
  [No_CAN3_BUS_OFF] -> PMM/62(No_CAN3_BUS_OFF)
  [DTC_clear_request] -> PMM/63(DTC_clear_request)
  [VPMM_PwrStaSW_enum] -> PMM/31(VPMM_PwrStaSW_enum)
  [VPMM_PowerSta_enum] -> PMM/30(VPMM_PowerSta_enum)
  [task_time_s] -> PMM/1(task_time_s)
  VINP_CAN3BusOff_flg/1 -> Logical Operator7/1
  VINP_CAN1BusOff_flg/1 -> Logical Operator6/1
  VPMM_PwrStaSW_enum/1 -> [VPMM_PwrStaSW_enum]
  VPMM_PowerSta_enum/1 -> [VPMM_PowerSta_enum]
  task_time_s/1 -> [task_time_s]
  PMM/54(VDDM_EDriveSysErrPMM_flg) -> [VDDM_EDriveSysErrPMM_flg]
  VPMM_DrivetrainSelect_enum/1 -> [VPMM_DrivetrainSelect_enum]
  VINP_LVBattDet12V_V/1 -> [VINP_LVBattDet12V_V]
  VINP_MCUWarnRNidec_enum/1 -> [VINP_MCUWarnRNidec_enum]
  VINP_MCUWarnFNidec_enum/1 -> [VINP_MCUWarnFNidec_enum]
  VINP_DCDCFaultSta_enum/1 -> [VINP_DCDCFaultSta_enum]
  TQD/35(VDDM_EDriveSysErrTQD_flg) -> [VDDM_EDriveSysErrTQD_flg]
  TQD/36(VDDM_EDriveSysErrShifterErr_flg) -> [VDDM_EDriveSysErrShifterErr_flg]
  TQD/37(VDDM_EngagePFail_flg) -> [VDDM_EngagePFail_flg]
  [VINP_LVBattDet12V_V] -> PMM/22(VINP_LVBattDet12V_V)
  Ground1/1 -> VDDM_EDriveSysErr_VCUErrTmp_flg/1  "VDDM_EDriveSysErr_VCUErrTmp_flg"
  [VDDM_LimpHomeActTmp_flg] -> VDDM_LimpHomeActTmp_flg/1  "VDDM_LimpHomeActTmp_flg"
  [VPMM_DrivetrainSelect_enum] -> PMM/34(VPMM_DrivetrainSelect_enum)
  [VPMM_DrivetrainSelect_enum] -> TQD/47(VPMM_DrivetrainSelect_enum)
  [VINP_BMSWarn4_flg] -> TQD/41(VINP_BMSWarn4_flg)
  [VINP_BMSWarn5_flg] -> TQD/42(VINP_BMSWarn5_flg)
  [VINP_BMSWarn6_flg] -> TQD/43(VINP_BMSWarn6_flg)
  [VINP_BMSWarn7_flg] -> TQD/44(VINP_BMSWarn7_flg)
  [VINP_BMSWarn8_flg] -> TQD/45(VINP_BMSWarn8_flg)
  [VINP_DCDCFaultSta_enum] -> TQD/46(VINP_DCDCFaultSta_enum)
  TQD/38(VDDM_VehMalfunLevelTmp_enum) -> [VDDM_VehMalfunLevelTmp_enum]
  TQD/39(VDDM_EPBLockTODTC_raw32) -> [VDDM_EPBLockTODTC_raw32]
  TQD/40(VDDM_EPBUnlockTODTC_raw32) -> [VDDM_EPBUnlockTODTC_raw32]
  TQD/41(VDDM_EPB1NoComDTC_raw32) -> [VDDM_EPB1NoComDTC_raw32]
  TQD/43(VDDM_EPB1CSErrDTC_raw32) -> [VDDM_EPB1CSErrDTC_raw32]
  TQD/42(VDDM_EPB1RCErrDTC_raw32) -> [VDDM_EPB1RCErrDTC_raw32]
  TQD/44(VDDM_EPBSigErrDTC_raw32) -> [VDDM_EPBSigErrDTC_raw32]
  TQD/45(VDDM_5vAPS1OoRCFS_flg) -> [VDDM_5vAPS1OoRCFS_flg]
  TQD/52(VDDM_Shifter1CSErrCFS_flg) -> [VDDM_Shifter1CSErrCFS_flg]
  TQD/51(VDDM_Shifter1RCErrCFS_flg) -> [VDDM_Shifter1RCErrCFS_flg]
  TQD/50(VDDM_Shifter1NoComCFS_flg) -> [VDDM_Shifter1NoComCFS_flg]
  TQD/49(VDDM_APSCorrErrCFS_flg) -> [VDDM_APSCorrErrCFS_flg]
  TQD/48(VDDM_APS2SigOoRCFS_flg) -> [VDDM_APS2SigOoRCFS_flg]
  TQD/47(VDDM_APS1SigOoRCFS_flg) -> [VDDM_APS1SigOoRCFS_flg]
  TQD/46(VDDM_5vAPS2OoRCFS_flg) -> [VDDM_5vAPS2OoRCFS_flg]
  TQD/53(VDDM_EPBSigErrCFS_flg) -> [VDDM_EPBSigErrCFS_flg]
  TQD/54(VDDM_EPB1NoComCFS_flg) -> [VDDM_EPB1NoComCFS_flg]
  TQD/56(VDDM_EPB1CSErrCFS_flg) -> [VDDM_EPB1CSErrCFS_flg]
  TQD/55(VDDM_EPB1RCErrCFS_flg) -> [VDDM_EPB1RCErrCFS_flg]
  TQD/57(VDDM_EPBLockTOCFS_flg) -> [VDDM_EPBLockTOCFS_flg]
  TQD/60(VDDM_RrMCUNTqErrCFS_flg) -> [VDDM_RrMCUNTqErrCFS_flg]
  TQD/59(VDDM_FrMCUNTqErrCFS_flg) -> [VDDM_FrMCUNTqErrCFS_flg]
  TQD/58(VDDM_EPBUnlockTOCFS_flg) -> [VDDM_EPBUnlockTOCFS_flg]
  [VTQD_GearActualPosn_enum] -> TQD/48(VTQD_GearActualPosn_enum)
  [VINP_EPBErrSta_enum] -> TQD/49(VINP_EPBErrSta_enum)
  [VINP_CANMsgValidEPB1_flg] -> TQD/50(VINP_CANMsgValidEPB1_flg)
  [VDDM_EPB1RCErr_flg] -> TQD/51(VDDM_EPB1RCErr_flg)
  [VDDM_EPB1CSErr_flg] -> TQD/52(VDDM_EPB1CSErr_flg)
  [VDHP_EAPS1BAD_flg] -> TQD/53(VDHP_EAPS1BAD_flg)
  [VDHP_EAPS2BAD_flg] -> TQD/54(VDHP_EAPS2BAD_flg)
  PMM/48(VDDM_VCUFLDoorSta_flg) -> [VDDM_VCUFLDoorSta_flg]
  PMM/49(VDDM_VCUFRDoorSta_flg) -> [VDDM_VCUFRDoorSta_flg]
  PMM/50(VDDM_VCURLDoorSta_flg) -> [VDDM_VCURLDoorSta_flg]
  PMM/51(VDDM_VCURRDoorSta_flg) -> [VDDM_VCURRDoorSta_flg]
  PMM/52(VDDM_VCUHoodSWSta_flg) -> [VDDM_VCUHoodSWSta_flg]
  PMM/53(VDDM_VCUTailgateSWSta_flg) -> [VDDM_VCUTailgateSWSta_flg]
  PMM/57(VDDM_HVRlyOpFail_flg) -> [VDDM_HVRlyOpFail_flg]
  PMM/58(VDDM_MCUActDisFail_flg) -> [VDDM_MCUActDisFail_flg]
  PMM/59(VDDM_C3BMS6CSCFS_flg) -> [VDDM_C3BMS6CSCFS_flg]
  PMM/60(VDDM_C3BMS6RCCFS_flg) -> [VDDM_C3BMS6RCCFS_flg]
  PMM/61(VDDM_C3BMS6LCCFS_flg) -> [VDDM_C3BMS6LCCFS_flg]
  PMM/62(VDDM_C3CCU2CSCFS_flg) -> [VDDM_C3CCU2CSCFS_flg]
  PMM/63(VDDM_C3CCU2LCCFS_flg) -> [VDDM_C3CCU2LCCFS_flg]
  PMM/64(VDDM_C3CCU2RCCFS_flg) -> [VDDM_C3CCU2RCCFS_flg]
  PMM/40(VDDM_LVInErrDTC_raw32) -> [VDDM_LVInErrDTC_raw32]
  PMM/65(VDDM_C3BMS1RCCFS_flg) -> [VDDM_C3BMS1RCCFS_flg]
  PMM/66(VDDM_C3BMS1CSCFS_flg) -> [VDDM_C3BMS1CSCFS_flg]
  PMM/67(VDDM_C3BMS1LCCFS_flg) -> [VDDM_C3BMS1LCCFS_flg]
  PMM/68(VDDM_C3CCU1RCCFS_flg) -> [VDDM_C3CCU1RCCFS_flg]
  PMM/69(VDDM_C3CCU1CSCFS_flg) -> [VDDM_C3CCU1CSCFS_flg]
  PMM/70(VDDM_C3CCU1LCCFS_flg) -> [VDDM_C3CCU1LCCFS_flg]
  PMM/71(VDDM_C1ABM1RCCFS_flg) -> [VDDM_C1ABM1RCCFS_flg]
  PMM/72(VDDM_C1ABM1CSCFS_flg) -> [VDDM_C1ABM1CSCFS_flg]
  PMM/73(VDDM_C1ABM1LCCFS_flg) -> [VDDM_C1ABM1LCCFS_flg]
  PMM/74(VDDM_Lv1ErrCFS_flg) -> [VDDM_Lv1ErrCFS_flg]
  PMM/75(VDDM_Lv2ErrCFS_flg) -> [VDDM_Lv2ErrCFS_flg]
  PMM/76(VDDM_Lv3ErrCFS_flg) -> [VDDM_Lv3ErrCFS_flg]
  PMM/77(VDDM_Lv4ErrCFS_flg) -> [VDDM_Lv4ErrCFS_flg]
  PMM/78(VDDM_IniLVLoCFS_flg) -> [VDDM_IniLVLoCFS_flg]
  PMM/79(VDDM_LVSupLoCFS_flg) -> [VDDM_LVSupLoCFS_flg]
  PMM/80(VDDM_LVSupHiCFS_flg) -> [VDDM_LVSupHiCFS_flg]
  PMM/81(VDDM_LVInErrCFS_flg) -> [VDDM_LVInErrCFS_flg]
  PMM/82(VDDM_HVB4PreCFS_flg) -> [VDDM_HVB4PreCFS_flg]
  PMM/83(VDDM_MCU4PreCFS_flg) -> [VDDM_MCU4PreCFS_flg]
  PMM/84(VDDM_DCDC4PreCFS_flg) -> [VDDM_DCDC4PreCFS_flg]
  PMM/85(VDDM_HVRlyCloCFS_flg) -> [VDDM_HVRlyCloCFS_flg]
  PMM/86(VDDM_BMSRdyCFS_flg) -> [VDDM_BMSRdyCFS_flg]
  PMM/87(VDDM_DCDCEnaCFS_flg) -> [VDDM_DCDCEnaCFS_flg]
  PMM/88(VDDM_HiLvSaChkCFS_flg) -> [VDDM_HiLvSaChkCFS_flg]
  PMM/89(VDDM_MidLvSaChkCFS_flg) -> [VDDM_MidLvSaChkCFS_flg]
  PMM/90(VDDM_MCUDisCFS_flg) -> [VDDM_MCUDisCFS_flg]
  PMM/91(VDDM_DCDCDisCFS_flg) -> [VDDM_DCDCDisCFS_flg]
  PMM/92(VDDM_HVRlyOpCFS_flg) -> [VDDM_HVRlyOpCFS_flg]
  PMM/93(VDDM_MCUActCFS_flg) -> [VDDM_MCUActCFS_flg]
  PMM/94(VDDM_OBC4PreCFS_flg) -> [VDDM_OBC4PreCFS_flg]
  PMM/95(VDDM_KeyAuthCFS_flg) -> [VDDM_KeyAuthCFS_flg]
  PMM/96(VDDM_ONtoRdyCFS_flg) -> [VDDM_ONtoRdyCFS_flg]
  PMM/97(VDDM_DrStSWCFS_flg) -> [VDDM_DrStSWCFS_flg]
  PMM/98(VDDM_FLDoorSWCFS_flg) -> [VDDM_FLDoorSWCFS_flg]
  PMM/99(VDDM_RLDoorSWCFS_flg) -> [VDDM_RLDoorSWCFS_flg]
  PMM/100(VDDM_FRDoorSWCFS_flg) -> [VDDM_FRDoorSWCFS_flg]
  PMM/101(VDDM_RRDoorSWCFS_flg) -> [VDDM_RRDoorSWCFS_flg]
  PMM/102(VDDM_HoodSWCFS_flg) -> [VDDM_HoodSWCFS_flg]
  PMM/103(VDDM_TailgaSWCFS_flg) -> [VDDM_TailgaSWCFS_flg]
  PMM/104(VDDM_BrkSWErrCFS_flg) -> [VDDM_BrkSWErrCFS_flg]
  PMM/105(VDDM_BrkSWNoBacCFS_flg) -> [VDDM_BrkSWNoBacCFS_flg]
  VMC_DDM/1(VDDM_FCM1NoComDTC_raw32) -> [VDDM_FCM1NoComDTC_raw32]
  VMC_DDM/2(VDDM_FCM1RCErrDTC_raw32) -> [VDDM_FCM1RCErrDTC_raw32]
  VMC_DDM/3(VDDM_FCM1CSErrDTC_raw32) -> [VDDM_FCM1CSErrDTC_raw32]
  VMC_DDM/4(VDDM_BMSSigErrDetDTC_raw32) -> [VDDM_BMSSigErrDetDTC_raw32]
  VMC_DDM/5(VDDM_FCMACCSigErrDetDTC_raw32) -> [VDDM_FCMACCSigErrDetDTC_raw32]
  VMC_DDM/6(VDDM_CCUSigErrDetDTC_raw32) -> [VDDM_CCUSigErrDetDTC_raw32]
  VMC_DDM/7(VDDM_ACCAccelCmdErrDetDTC_raw32) -> [VDDM_ACCAccelCmdErrDetDTC_raw32]
  VMC_DDM/8(VDDM_ESCSigErrDetDTC_raw32) -> [VDDM_ESCSigErrDetDTC_raw32]
  VMC_DDM/9(VDDM_ShifterSigErrDetDTC_raw32) -> [VDDM_ShifterSigErrDetDTC_raw32]
  VMC_DDM/10(VDDM_DrVCUNoComDTC_raw32) -> [VDDM_DrVCUNoComDTC_raw32]
  VMC_DDM/11(VDDM_FrVCUNoComDTC_raw32) -> [VDDM_FrVCUNoComDTC_raw32]
  VMC_DDM/12(VDDM_ZoneDrSigErrDetDTC_raw32) -> [VDDM_ZoneDrSigErrDetDTC_raw32]
  VMC_DDM/13(VDDM_ZoneFrSigErrDetDTC_raw32) -> [VDDM_ZoneFrSigErrDetDTC_raw32]
  VMC_DDM/14(VDDM_EPS1NoComDTC_raw32) -> [VDDM_EPS1NoComDTC_raw32]
  VMC_DDM/15(VDDM_EPS1RCErrDTC_raw32) -> [VDDM_EPS1RCErrDTC_raw32]
  VMC_DDM/16(VDDM_EPS1CSErrDTC_raw32) -> [VDDM_EPS1CSErrDTC_raw32]
  VMC_DDM/17(VDDM_EPSSigErrDTC_raw32) -> [VDDM_EPSSigErrDTC_raw32]
  VMC_DDM/18(VDDM_FrMCUSigErrDetDTC_raw32) -> [VDDM_FrMCUSigErrDetDTC_raw32]
  VMC_DDM/19(VDDM_RrMCUSigErrDetDTC_raw32) -> [VDDM_RrMCUSigErrDetDTC_raw32]
  VMC_DDM/20(VDDM_FCM1NoComCFS_flg) -> [VDDM_FCM1NoComCFS_flg]
  VMC_DDM/21(VDDM_FCM1RCErrCFS_flg) -> [VDDM_FCM1RCErrCFS_flg]
  VMC_DDM/22(VDDM_FCM1CSErrCFS_flg) -> [VDDM_FCM1CSErrCFS_flg]
  VMC_DDM/23(VDDM_BMSSigErrCFS_flg) -> [VDDM_BMSSigErrCFS_flg]
  VMC_DDM/24(VDDM_FCMACCSigErrCFS_flg) -> [VDDM_FCMACCSigErrCFS_flg]
  VMC_DDM/25(VDDM_CCUSigErrCFS_flg) -> [VDDM_CCUSigErrCFS_flg]
  VMC_DDM/26(VDDM_ACCAccelCmdErrCFS_flg) -> [VDDM_ACCAccelCmdErrCFS_flg]
  VMC_DDM/27(VDDM_ESCSigErrCFS_flg) -> [VDDM_ESCSigErrCFS_flg]
  VMC_DDM/28(VDDM_ShifterSigErrCFS_flg) -> [VDDM_ShifterSigErrCFS_flg]
  VMC_DDM/29(VDDM_DrVCUNoComCFS_flg) -> [VDDM_DrVCUNoComCFS_flg]
  VMC_DDM/30(VDDM_FrVCUNoComCFS_flg) -> [VDDM_FrVCUNoComCFS_flg]
  VMC_DDM/31(VDDM_ZoneDrSigErrCFS_flg) -> [VDDM_ZoneDrSigErrCFS_flg]
  VMC_DDM/32(VDDM_ZoneFrSigErrCFS_flg) -> [VDDM_ZoneFrSigErrCFS_flg]
  VMC_DDM/33(VDDM_EPS1NoComCFS_flg) -> [VDDM_EPS1NoComCFS_flg]
  VMC_DDM/34(VDDM_EPS1RCErrCFS_flg) -> [VDDM_EPS1RCErrCFS_flg]
  VMC_DDM/35(VDDM_EPS1CSErrCFS_flg) -> [VDDM_EPS1CSErrCFS_flg]
  VMC_DDM/36(VDDM_EPSSigErrCFS_flg) -> [VDDM_EPSSigErrCFS_flg]
  VMC_DDM/37(VDDM_FrMCUSigErrCFS_flg) -> [VDDM_FrMCUSigErrCFS_flg]
  VMC_DDM/38(VDDM_RrMCUSigErrCFS_flg) -> [VDDM_RrMCUSigErrCFS_flg]
  [No_CAN6_BUS_OFF] -> VMC_DDM/43(No_CAN6_BUS_OFF)
  [VTQD_ExternalTqAllow_flg] -> VMC_DDM/44(VTQD_ExternalTqAllow_flg)
  [VTQD_ExtDoorAllow_flg] -> VMC_DDM/45(VTQD_ExtDoorAllow_flg)
  [VINP_BMSWarn2_flg] -> VMC_DDM/46(VINP_BMSWarn2_flg)
  [VINP_BMSWarn1_flg] -> VMC_DDM/47(VINP_BMSWarn1_flg)
  [VDDM_Shifter1NoComCFS_flg] -> VMC_DDM/48(VDDM_Shifter1NoComCFS_flg)
  [VDDM_Shifter1RCErrCFS_flg] -> VMC_DDM/49(VDDM_Shifter1RCErrCFS_flg)
  [VDDM_Shifter1CSErrCFS_flg] -> VMC_DDM/50(VDDM_Shifter1CSErrCFS_flg)
  [VINP_ShifterFailsta_enum] -> VMC_DDM/51(VINP_ShifterFailsta_enum)
  [VTQD_GearActualPosn_enum] -> VMC_DDM/52(VTQD_GearActualPosn_enum)
  [VINP_HDDFailed_flg] -> VMC_DDM/54(VINP_HDDFailed_flg)
  [VINP_EBDFailed_flg] -> VMC_DDM/53(VINP_EBDFailed_flg)
  [VINP_ABSFailed_flg] -> VMC_DDM/55(VINP_ABSFailed_flg)
  [VINP_TCSFailed_flg] -> VMC_DDM/56(VINP_TCSFailed_flg)
  [VINP_ESCFailed_flg] -> VMC_DDM/57(VINP_ESCFailed_flg)
  [VINP_HBBFailed_flg] -> VMC_DDM/58(VINP_HBBFailed_flg)
  [VINP_PBAFailed_flg] -> VMC_DDM/59(VINP_PBAFailed_flg)
  [VINP_HSAFailed_flg] -> VMC_DDM/60(VINP_HSAFailed_flg)
  [VINP_AVHFailed_flg] -> VMC_DDM/61(VINP_AVHFailed_flg)
  [VINP_MCPressureV_flg] -> VMC_DDM/62(VINP_MCPressureV_flg)
  [VINP_BrkSwV_flg] -> VMC_DDM/63(VINP_BrkSwV_flg)
  [VINP_BrkPedalPosSta_flg] -> VMC_DDM/64(VINP_BrkPedalPosSta_flg)
  [VINP_LongAccelV_flg] -> VMC_DDM/65(VINP_LongAccelV_flg)
  [VINP_LatAccelV_flg] -> VMC_DDM/66(VINP_LatAccelV_flg)
  [VINP_YawRateV_flg] -> VMC_DDM/67(VINP_YawRateV_flg)
  [VINP_RFPulseCountV_flg] -> VMC_DDM/68(VINP_RFPulseCountV_flg)
  [VINP_RRPulseCountV_flg] -> VMC_DDM/69(VINP_RRPulseCountV_flg)
  [VINP_LFPulseCountV_flg] -> VMC_DDM/70(VINP_LFPulseCountV_flg)
  [VINP_LRPulseCountV_flg] -> VMC_DDM/71(VINP_LRPulseCountV_flg)
  [VINP_LRRawWhlSpeedV_flg] -> VMC_DDM/72(VINP_LRRawWhlSpeedV_flg)
  [VINP_RRRawWhlSpeedV_flg] -> VMC_DDM/73(VINP_RRRawWhlSpeedV_flg)
  [VINP_LFRawWhlSpeedV_flg] -> VMC_DDM/74(VINP_LFRawWhlSpeedV_flg)
  [VINP_RFRawWhlSpeedV_flg] -> VMC_DDM/75(VINP_RFRawWhlSpeedV_flg)
  [VINP_CANMsgValidZoneDrVCU_flg] -> VMC_DDM/76(VINP_CANMsgValidZoneDrVCU_flg)
  [VINP_CANMsgValidZoneFrVCU_flg] -> VMC_DDM/77(VINP_CANMsgValidZoneFrVCU_flg)
  [VINP_ZoneDrMalfunLevel_enum] -> VMC_DDM/78(VINP_ZoneDrMalfunLevel_enum)
  [ZoneFrMalfunLevel_enum] -> VMC_DDM/79(ZoneFrMalfunLevel_enum)
  [VINP_CANMsgValidEPS1_flg] -> VMC_DDM/80(VINP_CANMsgValidEPS1_flg)
  [VDDM_EPSRCErr_flg] -> VMC_DDM/81(VDDM_EPSRCErr_flg)
  [VDDM_EPSCSErr_flg] -> VMC_DDM/82(VDDM_EPSCSErr_flg)
  [VINP_SASV_flg] -> VMC_DDM/83(VINP_SASV_flg)
  [VPMM_DrivetrainSelect_enum] -> VMC_DDM/84(VPMM_DrivetrainSelect_enum)
  [VDDM_MCUNR1RCErrCFS_flg] -> PMM/70(VDDM_MCUNR1RCErrCFS_flg)
  [VDDM_MCUNR1CSErrCFS_flg] -> PMM/71(VDDM_MCUNR1CSErrCFS_flg)
  [VDDM_MCUNF1RCErrCFS_flg] -> PMM/72(VDDM_MCUNF1RCErrCFS_flg)
  [VDDM_MCUNF1CSErrCFS_flg] -> PMM/73(VDDM_MCUNF1CSErrCFS_flg)
  [VDDM_ESC1SigErr_flg] -> PMM/74(VDDM_ESC1SigErr_flg)
  [VDDM_ESC5SigErr_flg] -> PMM/75(VDDM_ESC5SigErr_flg)
  [VINP_ShifterFailsta_enum] -> PMM/76(VINP_ShifterFailsta_enum)
  [VDDM_Shifter1NoComCFS_flg] -> PMM/77(VDDM_Shifter1NoComCFS_flg)
  [VDDM_Shifter1RCErrCFS_flg] -> PMM/78(VDDM_Shifter1RCErrCFS_flg)
  [VDDM_Shifter1CSErrCFS_flg] -> PMM/79(VDDM_Shifter1CSErrCFS_flg)
  [No_CAN4_BUS_OFF] -> PMM/80(No_CAN4_BUS_OFF)
  [No_CAN4_BUS_OFF] -> VMC_DDM/42(No_CAN4_BUS_OFF)
  VINP_CAN4BusOff_flg/1 -> Logical Operator11/1
  [VINP_ZoneDrMalfunLevel_enum] -> PMM/81(VINP_ZoneDrMalfunLevel_enum)
  [VDDM_DrVCUNoComCFS_flg] -> PMM/82(VDDM_DrVCUNoComCFS_flg)
  [ZoneFrMalfunLevel_enum] -> PMM/83(ZoneFrMalfunLevel_enum)
  [VDDM_FrVCUNoComCFS_flg] -> PMM/84(VDDM_FrVCUNoComCFS_flg)
  [VDDM_AuxBattVolV_V] -> PMM/85(VDDM_AuxBattVolV_V)
  [VPMM_MCUDCBusMaxVolt_V] -> PMM/86(VPMM_MCUDCBusMaxVolt_V)
  VINP_BMSWarn3_flg/1 -> [VINP_BMSWarn3_flg]
  VINP_BMSWarn2_flg/1 -> [VINP_BMSWarn2_flg]
  VINP_BMSWarn1_flg/1 -> [VINP_BMSWarn1_flg]
  [VINP_BMSWarn2_flg] -> PMM/11(VINP_BMSWarn2_flg)
  [VINP_BMSWarn1_flg] -> PMM/10(VINP_BMSWarn1_flg)
  [VINP_BMSWarn3_flg] -> PMM/12(VINP_BMSWarn3_flg)
  [VINP_BMSWarn3_flg] -> VMC_DDM/17(VINP_BMSWarn3_flg)
  VMC_DDM/39(VDDM_ESC1SigErr_flg) -> [VDDM_ESC1SigErr_flg]
  VMC_DDM/40(VDDM_ESC5SigErr_flg) -> [VDDM_ESC5SigErr_flg]
  VINP_ShifterFailsta_enum/1 -> [VINP_ShifterFailsta_enum]
  No_CAN_BUS_OFF/1 -> Logical Operator12/1
  VINP_CAN6BusOff_flg/1 -> Logical Operator13/1
  [No_CAN_BUS_OFF] -> VMC_DDM/5(No_CAN_BUS_OFF)
  ZoneFrMalfunLevel_enum/1 -> [ZoneFrMalfunLevel_enum]
  VPMM_PowerUpState_enum/1 -> [VPMM_PowerUpState_enum]
  [VPMM_PowerUpState_enum] -> PMM/69(VPMM_PowerUpState_enum)
  VPMM_MCUDCBusMaxVolt_V/1 -> [VPMM_MCUDCBusMaxVolt_V]
  VTQD_GearActualPosn_enum/1 -> [VTQD_GearActualPosn_enum]
  VINP_EPBErrSta_enum/1 -> [VINP_EPBErrSta_enum]
  VINP_CANMsgValidEPB1_flg/1 -> [VINP_CANMsgValidEPB1_flg]
  VDDM_EPB1RCErr_flg/1 -> [VDDM_EPB1RCErr_flg]
  VDDM_EPB1CSErr_flg/1 -> [VDDM_EPB1CSErr_flg]
  VDHP_EAPS1BAD_flg/1 -> [VDHP_EAPS1BAD_flg]
  VDHP_EAPS2BAD_flg/1 -> [VDHP_EAPS2BAD_flg]
  [VDDM_FCM1CSErr_flg] -> VMC_DDM/4(VDDM_FCM1CSErr_flg)
  [VDDM_FCM1RCErr_flg] -> VMC_DDM/3(VDDM_FCM1RCErr_flg)
  [VINP_CANMsgValidFCM1_flg] -> VMC_DDM/2(VDDM_FCM1NoCom_flg)
  VINP_CANMsgValidFCM1_flg/1 -> [VINP_CANMsgValidFCM1_flg]
  VDDM_FCM1RCErr_flg/1 -> [VDDM_FCM1RCErr_flg]
  VDDM_FCM1CSErr_flg/1 -> [VDDM_FCM1CSErr_flg]
  [VINP_ADASACCSta_enum] -> VMC_DDM/7(VINP_ADASACCSta_enum)
  VINP_ADASACCSta_enum/1 -> [VINP_ADASACCSta_enum]
  VINP_ACCRequireAccel_mps2/1 -> [VINP_ACCRequireAccel_mps2]
  [VINP_ACCRequireAccel_mps2] -> VMC_DDM/32(VINP_ACCRequireAccel_mps2)
  VTQD_ExternalTqAllow_flg/1 -> [VTQD_ExternalTqAllow_flg]
  VTQD_ExtDoorAllow_flg/1 -> [VTQD_ExtDoorAllow_flg]
  VINP_EBDFailed_flg/1 -> [VINP_EBDFailed_flg]
  VINP_HDDFailed_flg/1 -> [VINP_HDDFailed_flg]
  VINP_ABSFailed_flg/1 -> [VINP_ABSFailed_flg]
  VINP_TCSFailed_flg/1 -> [VINP_TCSFailed_flg]
  VINP_ESCFailed_flg/1 -> [VINP_ESCFailed_flg]
  VINP_HBBFailed_flg/1 -> [VINP_HBBFailed_flg]
  VINP_BrkSwV_flg/1 -> [VINP_BrkSwV_flg]
  VINP_MCPressureV_flg/1 -> [VINP_MCPressureV_flg]
  VINP_AVHFailed_flg/1 -> [VINP_AVHFailed_flg]
  VINP_HSAFailed_flg/1 -> [VINP_HSAFailed_flg]
  VINP_PBAFailed_flg/1 -> [VINP_PBAFailed_flg]
  VINP_BrkPedalPosSta_flg/1 -> [VINP_BrkPedalPosSta_flg]
  VINP_LongAccelV_flg/1 -> [VINP_LongAccelV_flg]
  VINP_LatAccelV_flg/1 -> [VINP_LatAccelV_flg]
  VINP_YawRateV_flg/1 -> [VINP_YawRateV_flg]
  VINP_RFPulseCountV_flg/1 -> [VINP_RFPulseCountV_flg]
  VINP_RRPulseCountV_flg/1 -> [VINP_RRPulseCountV_flg]
  VINP_LFPulseCountV_flg/1 -> [VINP_LFPulseCountV_flg]
  VINP_LRPulseCountV_flg/1 -> [VINP_LRPulseCountV_flg]
  VINP_LRRawWhlSpeedV_flg/1 -> [VINP_LRRawWhlSpeedV_flg]
  VINP_RRRawWhlSpeedV_flg/1 -> [VINP_RRRawWhlSpeedV_flg]
  VINP_LFRawWhlSpeedV_flg/1 -> [VINP_LFRawWhlSpeedV_flg]
  VINP_RFRawWhlSpeedV_flg/1 -> [VINP_RFRawWhlSpeedV_flg]
  VINP_CANMsgValidEPS1_flg/1 -> [VINP_CANMsgValidEPS1_flg]
  VDDM_EPSRCErr_flg/1 -> [VDDM_EPSRCErr_flg]
  VDDM_EPSCSErr_flg/1 -> [VDDM_EPSCSErr_flg]
  VINP_SASV_flg/1 -> [VINP_SASV_flg]
  [VDDM_LVInErrDTC_raw32] -> VDDM_LVInErrDTC_raw32/1
  [VDDM_EPB1NoComDTC_raw32] -> VDDM_EPB1NoComDTC_raw32/1
  [VDDM_EPB1RCErrDTC_raw32] -> VDDM_EPB1RCErrDTC_raw32/1
  [VDDM_EPB1CSErrDTC_raw32] -> VDDM_EPB1CSErrDTC_raw32/1
  [VDDM_EPBSigErrDTC_raw32] -> VDDM_EPBSigErrDTC_raw32/1
  [VDDM_FCM1CSErrDTC_raw32] -> VDDM_FCM1CSErrDTC_raw32/1
  [VDDM_FCM1RCErrDTC_raw32] -> VDDM_FCM1RCErrDTC_raw32/1
  [VDDM_FCM1NoComDTC_raw32] -> VDDM_FCM1NoComDTC_raw32/1
  [VDDM_ESCSigErrDetDTC_raw32] -> VDDM_ESCSigErrDetDTC_raw32/1
  [VDDM_ShifterSigErrDetDTC_raw32] -> VDDM_ShifterSigErrDetDTC_raw32/1
  [VDDM_DrVCUNoComDTC_raw32] -> VDDM_DrVCUNoComDTC_raw32/1
  [VDDM_FrVCUNoComDTC_raw32] -> VDDM_FrVCUNoComDTC_raw32/1
  [VDDM_ZoneDrSigErrDetDTC_raw32] -> VDDM_ZoneDrSigErrDetDTC_raw32/1
  [VDDM_ZoneFrSigErrDetDTC_raw32] -> VDDM_ZoneFrSigErrDetDTC_raw32/1
  [VDDM_EPS1NoComDTC_raw32] -> VDDM_EPS1NoComDTC_raw32/1
  [VDDM_EPS1RCErrDTC_raw32] -> VDDM_EPS1RCErrDTC_raw32/1
  [VDDM_EPS1CSErrDTC_raw32] -> VDDM_EPS1CSErrDTC_raw32/1
  [VDDM_EPSSigErrDTC_raw32] -> VDDM_EPSSigErrDTC_raw32/1
  [VDDM_FCM1NoComCFS_flg] -> Chart/72(VDDM_FCM1NoComCFS_flg)
  [VDDM_FCM1RCErrCFS_flg] -> Chart/73(VDDM_FCM1RCErrCFS_flg)
  [VDDM_FCM1CSErrCFS_flg] -> Chart/74(VDDM_FCM1CSErrCFS_flg)
  [VDDM_BMSSigErrCFS_flg] -> Chart/75(VDDM_BMSSigErrCFS_flg)
  [VDDM_FCMACCSigErrCFS_flg] -> Chart/76(VDDM_FCMACCSigErrCFS_flg)
  [VDDM_CCUSigErrCFS_flg] -> Chart/77(VDDM_CCUSigErrCFS_flg)
  [VDDM_ACCAccelCmdErrCFS_flg] -> Chart/78(VDDM_ACCAccelCmdErrCFS_flg)
  [VDDM_ESCSigErrCFS_flg] -> Chart/79(VDDM_ESCSigErrCFS_flg)
  [VDDM_ShifterSigErrCFS_flg] -> Chart/80(VDDM_ShifterSigErrCFS_flg)
  [VDDM_FrVCUNoComCFS_flg] -> Chart/82(VDDM_FrVCUNoComCFS_flg)
  [VDDM_DrVCUNoComCFS_flg] -> Chart/81(VDDM_DrVCUNoComCFS_flg)
  [VDDM_ZoneDrSigErrCFS_flg] -> Chart/83(VDDM_ZoneDrSigErrCFS_flg)
  [VDDM_ZoneFrSigErrCFS_flg] -> Chart/84(VDDM_ZoneFrSigErrCFS_flg)
  Chart/1(VDDM_VehMalfunLevel_enum) -> Switch/1
  [VDDM_EPS1NoComCFS_flg] -> Chart/85(VDDM_EPS1NoComCFS_flg)
  [VDDM_EPS1RCErrCFS_flg] -> Chart/86(VDDM_EPS1RCErrCFS_flg)
  [VDDM_EPS1CSErrCFS_flg] -> Chart/87(VDDM_EPS1CSErrCFS_flg)
  [VDDM_EPSSigErrCFS_flg] -> Chart/88(VDDM_EPSSigErrCFS_flg)
  [VDDM_FrMCUSigErrCFS_flg] -> Chart/89(VDDM_FrMCUSigErrCFS_flg)
  [VDDM_RrMCUSigErrCFS_flg] -> Chart/90(VDDM_RrMCUSigErrCFS_flg)
  [VDDM_LVInErrCFS_flg] -> Chart/42(VDDM_LVInErrCFS_flg)
  [VDDM_EPB1NoComCFS_flg] -> Chart/91(VDDM_EPB1NoComCFS_flg)
  [VDDM_EPB1RCErrCFS_flg] -> Chart/92(VDDM_EPB1RCErrCFS_flg)
  [VDDM_EPB1CSErrCFS_flg] -> Chart/93(VDDM_EPB1CSErrCFS_flg)
  [VDDM_EPBSigErrCFS_flg] -> Chart/94(VDDM_EPBSigErrCFS_flg)
  [VDDM_FrMCUNTqErrCFS_flg] -> Chart/95(VDDM_FrMCUNTqErrCFS_flg)
  [VDDM_RrMCUNTqErrCFS_flg] -> Chart/96(VDDM_RrMCUNTqErrCFS_flg)
  Switch/1 -> [VDDM_VehMalfunLevel_enum]  "VDDM_VehMalfunLevel_enum"
  VMC_DDM/41(VDDM_EDriveSysErrVCUErrVMC_flg) -> [VDDM_EDriveSysErrVCUErrVMC_flg]
  VINP_CANMsgValidZoneDrVCU_flg/1 -> [VINP_CANMsgValidZoneDrVCU_flg]
  VINP_CANMsgValidZoneFrVCU_flg/1 -> [VINP_CANMsgValidZoneFrVCU_flg]
  [VDDM_VehMalfunLevel_enum] -> Relational Operator/1
  Constant20/1 -> Relational Operator/2
  Relational Operator/1 -> Switch1/2
  Constant2/1 -> Switch1/3
  Constant3/1 -> Switch1/1
  Constant4/1 -> Switch2/2
  Switch8/1 -> [VDDM_LimpHomeActTmp_flg]  "VDDM_LimpHomeActTmp_flg"
  [VDDM_5vAPS1OoRCFS_flg] -> Enabled Subsystem/1(VDDM_5vAPS1OoRCFS_flg)
  [VDDM_5vAPS2OoRCFS_flg] -> Enabled Subsystem/2(VDDM_5vAPS2OoRCFS_flg)
  [VDDM_BMSRdyCFS_flg] -> Enabled Subsystem/3(VDDM_BMSRdyCFS_flg)
  [VDDM_BrkSWNoBacCFS_flg] -> Enabled Subsystem/5(VDDM_BrkSWNoBacCFS_flg)
  [VDDM_BrkSWErrCFS_flg] -> Enabled Subsystem/4(VDDM_BrkSWErrCFS_flg)
  [VDDM_C1ABM1CSCFS_flg] -> Enabled Subsystem/6(VDDM_C1ABM1CSCFS_flg)
  [VDDM_C1ABM1LCCFS_flg] -> Enabled Subsystem/7(VDDM_C1ABM1LCCFS_flg)
  [VDDM_C1ABM1RCCFS_flg] -> Enabled Subsystem/8(VDDM_C1ABM1RCCFS_flg)
  [VDDM_C3BMS1CSCFS_flg] -> Enabled Subsystem/9(VDDM_C3BMS1CSCFS_flg)
  [VDDM_C3BMS1LCCFS_flg] -> Enabled Subsystem/10(VDDM_C3BMS1LCCFS_flg)
  [VDDM_C3BMS1RCCFS_flg] -> Enabled Subsystem/11(VDDM_C3BMS1RCCFS_flg)
  [VDDM_C3BMS6CSCFS_flg] -> Enabled Subsystem/12(VDDM_C3BMS6CSCFS_flg)
  [VDDM_C3BMS6LCCFS_flg] -> Enabled Subsystem/13(VDDM_C3BMS6LCCFS_flg)
  [VDDM_C3BMS6RCCFS_flg] -> Enabled Subsystem/14(VDDM_C3BMS6RCCFS_flg)
  [VDDM_C3CCU1CSCFS_flg] -> Enabled Subsystem/15(VDDM_C3CCU1CSCFS_flg)
  [VDDM_C3CCU1LCCFS_flg] -> Enabled Subsystem/16(VDDM_C3CCU1LCCFS_flg)
  [VDDM_C3CCU1RCCFS_flg] -> Enabled Subsystem/17(VDDM_C3CCU1RCCFS_flg)
  [VDDM_C3CCU2CSCFS_flg] -> Enabled Subsystem/18(VDDM_C3CCU2CSCFS_flg)
  [VDDM_C3CCU2LCCFS_flg] -> Enabled Subsystem/19(VDDM_C3CCU2LCCFS_flg)
  [VDDM_C3CCU2RCCFS_flg] -> Enabled Subsystem/20(VDDM_C3CCU2RCCFS_flg)
  [VDDM_DCDC4PreCFS_flg] -> Enabled Subsystem/21(VDDM_DCDC4PreCFS_flg)
  [VDDM_DCDCDisCFS_flg] -> Enabled Subsystem/22(VDDM_DCDCDisCFS_flg)
  [VDDM_DCDCEnaCFS_flg] -> Enabled Subsystem/23(VDDM_DCDCEnaCFS_flg)
  [VDDM_DrStSWCFS_flg] -> Enabled Subsystem/24(VDDM_DrStSWCFS_flg)
  [VDDM_EPBLockTOCFS_flg] -> Enabled Subsystem/25(VDDM_EPBLockTOCFS_flg)
  [VDDM_EPBUnlockTOCFS_flg] -> Enabled Subsystem/26(VDDM_EPBUnlockTOCFS_flg)
  [VDDM_ESC1CSErrCFS_flg] -> Enabled Subsystem/27(VDDM_ESC1CSErrCFS_flg)
  [VDDM_ESC1NoComCFS_flg] -> Enabled Subsystem/28(VDDM_ESC1NoComCFS_flg)
  [VDDM_ESC1RCErrCFS_flg] -> Enabled Subsystem/29(VDDM_ESC1RCErrCFS_flg)
  [VDDM_ESC5CSErrCFS_flg] -> Enabled Subsystem/30(VDDM_ESC5CSErrCFS_flg)
  [VDDM_ESC5NoComCFS_flg] -> Enabled Subsystem/31(VDDM_ESC5NoComCFS_flg)
  [VDDM_IniLVLoCFS_flg] -> Enabled Subsystem/39(VDDM_IniLVLoCFS_flg)
  [VDDM_HiLvSaChkCFS_flg] -> Enabled Subsystem/38(VDDM_HiLvSaChkCFS_flg)
  [VDDM_HVRlyOpCFS_flg] -> Enabled Subsystem/37(VDDM_HVRlyOpCFS_flg)
  [VDDM_HVRlyCloCFS_flg] -> Enabled Subsystem/36(VDDM_HVRlyCloCFS_flg)
  [VDDM_HVB4PreCFS_flg] -> Enabled Subsystem/35(VDDM_HVB4PreCFS_flg)
  [VDDM_ESC5RCErrCFS_flg] -> Enabled Subsystem/32(VDDM_ESC5RCErrCFS_flg)
  [VDDM_FLDoorSWCFS_flg] -> Enabled Subsystem/33(VDDM_FLDoorSWCFS_flg)
  [VDDM_FRDoorSWCFS_flg] -> Enabled Subsystem/34(VDDM_FRDoorSWCFS_flg)
  [VDDM_KeyAuthCFS_flg] -> Enabled Subsystem/40(VDDM_KeyAuthCFS_flg)
  [VDDM_MCUDisCFS_flg] -> Enabled Subsystem/50(VDDM_MCUDisCFS_flg)
  [VDDM_MCU4PreCFS_flg] -> Enabled Subsystem/48(VDDM_MCU4PreCFS_flg)
  [VDDM_MCUActCFS_flg] -> Enabled Subsystem/49(VDDM_MCUActCFS_flg)
  [VDDM_Lv4ErrCFS_flg] -> Enabled Subsystem/47(VDDM_Lv4ErrCFS_flg)
  [VDDM_Lv3ErrCFS_flg] -> Enabled Subsystem/46(VDDM_Lv3ErrCFS_flg)
  [VDDM_Lv2ErrCFS_flg] -> Enabled Subsystem/45(VDDM_Lv2ErrCFS_flg)
  [VDDM_Lv1ErrCFS_flg] -> Enabled Subsystem/44(VDDM_Lv1ErrCFS_flg)
  [VDDM_LVSupLoCFS_flg] -> Enabled Subsystem/43(VDDM_LVSupLoCFS_flg)
  [VDDM_LVSupHiCFS_flg] -> Enabled Subsystem/42(VDDM_LVSupHiCFS_flg)
  [VDDM_LVInErrCFS_flg] -> Enabled Subsystem/41(VDDM_LVInErrCFS_flg)
  [VDDM_MCUNF1CSErrCFS_flg] -> Enabled Subsystem/51(VDDM_MCUNF1CSErrCFS_flg)
  [VDDM_MCUNF1NoComCFS_flg] -> Enabled Subsystem/52(VDDM_MCUNF1NoComCFS_flg)
  [VDDM_MCUNF1RCErrCFS_flg] -> Enabled Subsystem/53(VDDM_MCUNF1RCErrCFS_flg)
  [VDDM_MCUNR1CSErrCFS_flg] -> Enabled Subsystem/54(VDDM_MCUNR1CSErrCFS_flg)
  [VDDM_MCUNR1NoComCFS_flg] -> Enabled Subsystem/55(VDDM_MCUNR1NoComCFS_flg)
  [VDDM_MCUNR1RCErrCFS_flg] -> Enabled Subsystem/56(VDDM_MCUNR1RCErrCFS_flg)
  [VDDM_MidLvSaChkCFS_flg] -> Enabled Subsystem/57(VDDM_MidLvSaChkCFS_flg)
  [VDDM_OBC4PreCFS_flg] -> Enabled Subsystem/58(VDDM_OBC4PreCFS_flg)
  [VDDM_ONtoRdyCFS_flg] -> Enabled Subsystem/59(VDDM_ONtoRdyCFS_flg)
  [VDDM_RLDoorSWCFS_flg] -> Enabled Subsystem/60(VDDM_RLDoorSWCFS_flg)
  [VDDM_Shifter1CSErrCFS_flg] -> Enabled Subsystem/62(VDDM_Shifter1CSErrCFS_flg)
  [VDDM_Shifter1NoComCFS_flg] -> Enabled Subsystem/63(VDDM_Shifter1NoComCFS_flg)
  [VDDM_RRDoorSWCFS_flg] -> Enabled Subsystem/61(VDDM_RRDoorSWCFS_flg)
  [VDDM_Shifter1RCErrCFS_flg] -> Enabled Subsystem/64(VDDM_Shifter1RCErrCFS_flg)
  [VDDM_HoodSWCFS_flg] -> Enabled Subsystem/65(VDDM_HoodSWCFS_flg)
  [VDDM_TailgaSWCFS_flg] -> Enabled Subsystem/66(VDDM_TailgaSWCFS_flg)
  [VINP_ZoneDrMalfunLevel_enum] -> Enabled Subsystem/67(VINP_ZoneDrMalfunLevel_enum)
  [ZoneFrMalfunLevel_enum] -> Enabled Subsystem/68(ZoneFrMalfunLevel_enum)
  [VDDM_RrMCUNTqErrCFS_flg] -> Enabled Subsystem/96(VDDM_RrMCUNTqErrCFS_flg)
  [VDDM_FrMCUNTqErrCFS_flg] -> Enabled Subsystem/95(VDDM_FrMCUNTqErrCFS_flg)
  [VDDM_EPBSigErrCFS_flg] -> Enabled Subsystem/94(VDDM_EPBSigErrCFS_flg)
  [VDDM_EPB1CSErrCFS_flg] -> Enabled Subsystem/93(VDDM_EPB1CSErrCFS_flg)
  [VDDM_EPS1NoComCFS_flg] -> Enabled Subsystem/85(VDDM_EPS1NoComCFS_flg)
  [VDDM_EPS1RCErrCFS_flg] -> Enabled Subsystem/86(VDDM_EPS1RCErrCFS_flg)
  [VDDM_EPS1CSErrCFS_flg] -> Enabled Subsystem/87(VDDM_EPS1CSErrCFS_flg)
  [VDDM_EPSSigErrCFS_flg] -> Enabled Subsystem/88(VDDM_EPSSigErrCFS_flg)
  [VDDM_FrMCUSigErrCFS_flg] -> Enabled Subsystem/89(VDDM_FrMCUSigErrCFS_flg)
  [VDDM_RrMCUSigErrCFS_flg] -> Enabled Subsystem/90(VDDM_RrMCUSigErrCFS_flg)
  [VDDM_EPB1NoComCFS_flg] -> Enabled Subsystem/91(VDDM_EPB1NoComCFS_flg)
  [VDDM_EPB1RCErrCFS_flg] -> Enabled Subsystem/92(VDDM_EPB1RCErrCFS_flg)
  [VDDM_ESCSigErrCFS_flg] -> Enabled Subsystem/79(VDDM_ESCSigErrCFS_flg)
  [VDDM_ShifterSigErrCFS_flg] -> Enabled Subsystem/80(VDDM_ShifterSigErrCFS_flg)
  [VDDM_DrVCUNoComCFS_flg] -> Enabled Subsystem/81(VDDM_DrVCUNoComCFS_flg)
  [VDDM_FrVCUNoComCFS_flg] -> Enabled Subsystem/82(VDDM_FrVCUNoComCFS_flg)
  [VDDM_ZoneFrSigErrCFS_flg] -> Enabled Subsystem/84(VDDM_ZoneFrSigErrCFS_flg)
  [VDDM_ZoneDrSigErrCFS_flg] -> Enabled Subsystem/83(VDDM_ZoneDrSigErrCFS_flg)
  [VDDM_ACCAccelCmdErrCFS_flg] -> Enabled Subsystem/78(VDDM_ACCAccelCmdErrCFS_flg)
  [VDDM_CCUSigErrCFS_flg] -> Enabled Subsystem/77(VDDM_CCUSigErrCFS_flg)
  [VDDM_FCMACCSigErrCFS_flg] -> Enabled Subsystem/76(VDDM_FCMACCSigErrCFS_flg)
  [VDDM_BMSSigErrCFS_flg] -> Enabled Subsystem/75(VDDM_BMSSigErrCFS_flg)
  [VDDM_FCM1CSErrCFS_flg] -> Enabled Subsystem/74(VDDM_FCM1CSErrCFS_flg)
  [VDDM_FCM1RCErrCFS_flg] -> Enabled Subsystem/73(VDDM_FCM1RCErrCFS_flg)
  [VDDM_FCM1NoComCFS_flg] -> Enabled Subsystem/72(VDDM_FCM1NoComCFS_flg)
  [VDDM_APSCorrErrCFS_flg] -> Enabled Subsystem/71(VDDM_APSCorrErrCFS_flg)
  [VDDM_APS2SigOoRCFS_flg] -> Enabled Subsystem/70(VDDM_APS2SigOoRCFS_flg)
  [VDDM_APS1SigOoRCFS_flg] -> Enabled Subsystem/69(VDDM_APS1SigOoRCFS_flg)
  Enabled Subsystem/1(VDDM_DTCDetect_enum) -> [VDDM_DTCDetect_enum]
  [VDDM_DTCDetect_enum] -> VDDM_DTCDetect_enum/1
  Constant5/1 -> Switch3/3
  Constant7/1 -> Relational Operator1/2
  [VDDM_VehMalfunLevelTmp_enum] -> Relational Operator1/1
  Relational Operator1/1 -> Switch3/2
  Constant8/1 -> Switch3/1
  Switch3/1 -> Switch2/3
  Switch1/1 -> Switch2/1
  From514/1 -> Logical Operator1/3
  From515/1 -> Logical Operator1/2
  From516/1 -> Logical Operator1/1
  From206/1 -> Relational Operator2/1
  Relational Operator2/1 -> Logical Operator1/4
  Constant11/1 -> Relational Operator2/2
  TQD/61(VDDM_DisengagePFail_flg) -> [VDDM_DisengagePFail_flg]
  Constant12/1 -> Relational Operator3/2
  [VDDM_VehMalfunLevelTmp_enum] -> Relational Operator3/1
  Switch4/1 -> [VDDM_VCURAPSErrLv3_flg]  "VDDM_VCURAPSErrLv3_flg"
  Switch5/1 -> [VDDM_VCURAPSErrLv2_flg]  "VDDM_VCURAPSErrLv2_flg"
  [VDDM_DisengagePFail_flg] -> VDDM_DisengagePFail_flg/1
  [VDDM_VCURAPSErrLv2_flg] -> VDDM_VCURAPSErrLv2_flg/1
  [VDDM_VCURAPSErrLv3_flg] -> VDDM_VCURAPSErrLv3_flg/1
  [VDDM_EngagePFail_flg] -> VDDM_EngagePFail_flg/1
  VDHP_EAPS12RangeSta_enum/1 -> [VDHP_EAPS12RangeSta_enum]
  [VDDM_EDriveSysErrShifterErr_flg] -> VDDM_EDriveSysErrShifterErr_flg/1
  Constant13/1 -> Switch6/2
  [VDDM_VehMalfunLevel_enum] -> Switch6/1
  [VDDM_VehMalfunLevelTmp_enum] -> Switch6/3
  Switch6/1 -> Data Type Conversion1/1
  [VINP_CANMsgValidABM1_flg] -> PMM/2(VINP_CANMsgValidABM1_flg)
  [VINP_BrkPedalPosSta_enum] -> PMM/3(VINP_BrkPedalPosSta_enum)
  [VINP_BrkSWSta_flg] -> PMM/5(VINP_BrkSWSta_flg)
  [VINP_BrkPedalPos_pct] -> PMM/4(VINP_BrkPedalPos_pct)
  VINP_CANMsgValidABM1_flg/1 -> [VINP_CANMsgValidABM1_flg]
  VINP_BrkPedalPosSta_enum/1 -> [VINP_BrkPedalPosSta_enum]
  VINP_BrkPedalPos_pct/1 -> [VINP_BrkPedalPos_pct]
  VINP_BrkSWSta_flg/1 -> [VINP_BrkSWSta_flg]
  VINP_VehSpeed_kph/1 -> [VINP_VehSpeed_kph]
  [VDDM_C1ABM1RCChk_flg] -> PMM/48(VDDM_C1ABM1RCChk_flg)
  [VDDM_C1ABM1CSChk_flg] -> PMM/49(VDDM_C1ABM1CSChk_flg)
  VDDM_C1ABM1RCChk_flg/1 -> [VDDM_C1ABM1RCChk_flg]
  VDDM_C1ABM1CSChk_flg/1 -> [VDDM_C1ABM1CSChk_flg]
  [VINP_CANMsgValidBMS1_flg] -> PMM/6(VINP_CANMsgValidBMS1_flg)
  [VINP_CANMsgValidBMS6_flg] -> PMM/7(VINP_CANMsgValidBMS6_flg)
  [VINP_CANMsgValidCCU1_flg] -> PMM/8(VINP_CANMsgValidCCU1_flg)
  [VINP_CANMsgValidCCU2_flg] -> PMM/9(VINP_CANMsgValidCCU2_flg)
  VINP_CANMsgValidBMS1_flg/1 -> [VINP_CANMsgValidBMS1_flg]
  VINP_CANMsgValidBMS6_flg/1 -> [VINP_CANMsgValidBMS6_flg]
  VINP_CANMsgValidCCU1_flg/1 -> [VINP_CANMsgValidCCU1_flg]
  VINP_CANMsgValidCCU2_flg/1 -> [VINP_CANMsgValidCCU2_flg]
  [VINP_OBCFaultSta_enum] -> PMM/19(VINP_OBCFaultSta_enum)
  VINP_OBCFaultSta_enum/1 -> [VINP_OBCFaultSta_enum]
  [VINP_BMSREADY_flg] -> PMM/23(VINP_BMSREADY_flg)
  [VINP_HVBattReady4Pre_enum] -> PMM/24(VINP_HVBattReady4Pre_enum)
  [VINP_HVBContactorSta_flg] -> PMM/25(VINP_HVBContactorSta_flg)
  [VINP_DCDCReady4Pre_flg] -> PMM/26(VINP_DCDCReady4Pre_flg)
  [VINP_DCDCEnabled_flg] -> PMM/27(VINP_DCDCEnabled_flg)
  VINP_BMSREADY_flg/1 -> [VINP_BMSREADY_flg]
  VINP_HVBattReady4Pre_enum/1 -> [VINP_HVBattReady4Pre_enum]
  VINP_HVBContactorSta_flg/1 -> [VINP_HVBContactorSta_flg]
  VINP_DCDCReady4Pre_flg/1 -> [VINP_DCDCReady4Pre_flg]
  VINP_DCDCEnabled_flg/1 -> [VINP_DCDCEnabled_flg]
  [VDDM_C3BMS6RCChk_flg] -> PMM/40(VDDM_C3BMS6RCChk_flg)
  [VDDM_C3BMS6CSChk_flg] -> PMM/41(VDDM_C3BMS6CSChk_flg)
  [VDDM_C3BMS1RCChk_flg] -> PMM/42(VDDM_C3BMS1RCChk_flg)
  [VDDM_C3BMS1CSChk_flg] -> PMM/43(VDDM_C3BMS1CSChk_flg)
  [VDDM_C3CCU1RCChk_flg] -> PMM/44(VDDM_C3CCU1RCChk_flg)
  [VDDM_C3CCU1CSChk_flg] -> PMM/45(VDDM_C3CCU1CSChk_flg)
  [VDDM_C3CCU2RCChk_flg] -> PMM/46(VDDM_C3CCU2RCChk_flg)
  [VDDM_C3CCU2CSChk_flg] -> PMM/47(VDDM_C3CCU2CSChk_flg)
  VDDM_C3BMS6RCChk_flg/1 -> [VDDM_C3BMS6RCChk_flg]
  VDDM_C3BMS6CSChk_flg/1 -> [VDDM_C3BMS6CSChk_flg]
  VDDM_C3BMS1RCChk_flg/1 -> [VDDM_C3BMS1RCChk_flg]
  VDDM_C3BMS1CSChk_flg/1 -> [VDDM_C3BMS1CSChk_flg]
  VDDM_C3CCU1RCChk_flg/1 -> [VDDM_C3CCU1RCChk_flg]
  VDDM_C3CCU1CSChk_flg/1 -> [VDDM_C3CCU1CSChk_flg]
  VDDM_C3CCU2RCChk_flg/1 -> [VDDM_C3CCU2RCChk_flg]
  VDDM_C3CCU2CSChk_flg/1 -> [VDDM_C3CCU2CSChk_flg]
  [VINP_CANMsgValidBMS5_flg] -> PMM/28(VINP_CANMsgValidBMS5_flg)
  VINP_CANMsgValidBMS5_flg/1 -> [VINP_CANMsgValidBMS5_flg]
  [VPMM_PowerUpFault_enum] -> PMM/32(VPMM_PowerUpFault_enum)
  [VPMM_PowerDownFault_enum] -> PMM/33(VPMM_PowerDownFault_enum)
  VPMM_PowerUpFault_enum/1 -> [VPMM_PowerUpFault_enum]
  VPMM_PowerDownFault_enum/1 -> [VPMM_PowerDownFault_enum]
  [VPMM_SafetyChkHLv_flg] -> PMM/35(VPMM_SafetyChkHLv_flg)
  [VPMM_SafetyChkMLv_flg] -> PMM/36(VPMM_SafetyChkMLv_flg)
  [VPMM_HVChrgPreActionErrSta_enum] -> PMM/37(VPMM_HVChrgPreActionErrSta_enum)
  [VPMM_MCUReady_flg] -> PMM/38(VPMM_MCUReady_flg)
  [VPMM_MCUReady4Pre_flg] -> PMM/39(VPMM_MCUReady4Pre_flg)
  VPMM_SafetyChkHLv_flg/1 -> [VPMM_SafetyChkHLv_flg]
  VPMM_SafetyChkMLv_flg/1 -> [VPMM_SafetyChkMLv_flg]
  VPMM_HVChrgPreActionErrSta_enum/1 -> [VPMM_HVChrgPreActionErrSta_enum]
  VPMM_MCUReady_flg/1 -> [VPMM_MCUReady_flg]
  VPMM_MCUReady4Pre_flg/1 -> [VPMM_MCUReady4Pre_flg]
  [VINP_BrakeSWGPIO_flg] -> PMM/50(VINP_BrakeSWGPIO_flg)
  [VINP_BrakeLampSW_flg] -> PMM/51(VINP_BrakeLampSW_flg)
  [VINP_DrStSW] -> PMM/52(VINP_DrStSW)
  [VINP_FLAJARSW] -> PMM/53(VINP_FLAJARSW)
  [VINP_FRAJARSW] -> PMM/54(VINP_FRAJARSW)
  [VINP_RLAJARSW] -> PMM/55(VINP_RLAJARSW)
  [VINP_RRAJARSW] -> PMM/56(VINP_RRAJARSW)
  [VINP_HoodSW] -> PMM/57(VINP_HoodSW)
  [VINP_TailgaSW] -> PMM/58(VINP_TailgaSW)
  VINP_BrakeSWGPIO_flg/1 -> [VINP_BrakeSWGPIO_flg]
  VINP_BrakeLampSW_flg/1 -> [VINP_BrakeLampSW_flg]
  VINP_DrStSW/1 -> [VINP_DrStSW]
  VINP_FLAJARSW/1 -> [VINP_FLAJARSW]
  VINP_FRAJARSW/1 -> [VINP_FRAJARSW]
  VINP_RLAJARSW/1 -> [VINP_RLAJARSW]
  VINP_RRAJARSW/1 -> [VINP_RRAJARSW]
  VINP_HoodSW/1 -> [VINP_HoodSW]
  VINP_TailgaSW/1 -> [VINP_TailgaSW]
  [VINP_AccelPedal2Vol_V] -> TQD/3(VINP_AccelPedal2Vol_V)
  [VINP_AccelPedal1Vol_V] -> TQD/2(VINP_AccelPedal1Vol_V)
  VINP_AccelPedal1Vol_V/1 -> [VINP_AccelPedal1Vol_V]
  VINP_AccelPedal2Vol_V/1 -> [VINP_AccelPedal2Vol_V]
  [VDKC_DKCAuthSta_enum] -> PMM/59(VDKC_DKCAuthSta_enum)
  [VINP_AllowMovThd_OTA_enum] -> PMM/60(VINP_AllowMovThd_OTA_enum)
  VDKC_DKCAuthSta_enum/1 -> [VDKC_DKCAuthSta_enum]
  VINP_AllowMovThd_OTA_enum/1 -> [VINP_AllowMovThd_OTA_enum]
  [VINP_DrStdAErrSta_enum] -> PMM/29(VINP_DrStdAErrSta_enum)
  VINP_DrStdAErrSta_enum/1 -> [VINP_DrStdAErrSta_enum]
  [VVMC_ADASActive_flg] -> VMC_DDM/31(VVMC_ADASActive_flg)
  VVMC_ADASActive_flg/1 -> [VVMC_ADASActive_flg]
  [VINP_ZoneSpdCtrlMode_enum] -> VMC_DDM/39(VINP_ZoneSpdCtrlMode_enum)
  VINP_ZoneSpdCtrlMode_enum/1 -> [VINP_ZoneSpdCtrlMode_enum]
  Relational Operator4/1 -> Data Type Conversion/1
  [VDDM_EDriveSysErrVCUErr_flg] -> VDDM_EDriveSysErrVCUErr_flg/1
  [VDDM_C3BMS1LCCFS_flg] -> TQD/55(VDDM_C3BMS1LCCFS_flg)
  VINP_CANMsgValidDKC2_flg/1 -> [VINP_CANMsgValidDKC2_flg]
  VINP_CANMsgValidDKC1_flg/1 -> [VINP_CANMsgValidDKC1_flg]
  [VINP_CANMsgValidDKC1_flg] -> PMM/87(VINP_CANMsgValidDKC1_flg)
  [VINP_CANMsgValidDKC2_flg] -> PMM/88(VINP_CANMsgValidDKC2_flg)
  [No_CAN1_BUS_OFF] -> Logical Operator3/1
  Logical Operator3/1 -> Logical Operator/4
  PMM/106(VDDM_PMMBattErr_flg) -> [VDDM_PMMBattErr_flg]
  [VDDM_PMMBattErr_flg] -> VDDM_PMMBattErr_flg/1
  Constant36/1 -> Equal14/2
  From595/1 -> Equal14/1
  From594/1 -> Logical Operator4/1
  Switch9/1 -> [VDDM_LVSysErrPwrOutErr_flg]  "VDDM_LVSysErrPwrOutErr_flg"
  [VDDM_LVSysErrPwrOutErr_flg] -> VDDM_LVSysErrPwrOutErr_flg/1
  TQD/62(VDDM_Shifter1Err_flg) -> [VDDM_Shifter1Err_flg]
  TQD/63(VDDM_EPB1Err_flg) -> [VDDM_EPB1Err_flg]
  [VDDM_Shifter1Err_flg] -> Logical Operator/3
  [VDDM_EPBUnlockTOCFS_flg] -> Logical Operator/2
  [VDDM_ESCSigErrCFS_flg] -> Logical Operator9/3
  Logical Operator10/1 -> Logical Operator8/1
  [VDDM_ESC5Err_flg] -> Logical Operator9/2
  Logical Operator9/1 -> Logical Operator10/1
  [VDDM_ESC1Err_flg] -> Logical Operator9/1
  Logical Operator8/1 -> Logical Operator/1
  Relational Operator3/1 -> Logical Operator8/2
  [VDDM_EPB1Err_flg] -> Logical Operator2/1
  [VDDM_EPBSigErrCFS_flg] -> Logical Operator2/2
  [VDDM_EPBLockTOCFS_flg] -> Logical Operator2/3
  [VDDM_ESC1Err_flg] -> Logical Operator2/4
  [VDDM_ESCSigErrCFS_flg] -> Logical Operator2/6
  [VDDM_ESC5Err_flg] -> Logical Operator2/5
  [VVMC_APSActive_flg] -> TQD/57(VVMC_APSActive_flg)
  [VDDM_VCURAPSErrLv2_flg] -> TQD/56(VDDM_VCURAPSErrLv2_flg)
  VVMC_APSActive_flg/1 -> [VVMC_APSActive_flg]
  TQD/64(VDDM_ESC5Err_flg) -> [VDDM_ESC5Err_flg]
  TQD/65(VDDM_ESC1Err_flg) -> [VDDM_ESC1Err_flg]
  Logical Operator5/1 -> Logical Operator4/2
  Equal14/1 -> Logical Operator5/2
  From538/1 -> Logical Operator5/1
  Logical Operator6/1 -> [No_CAN1_BUS_OFF]
  Logical Operator7/1 -> [No_CAN3_BUS_OFF]
  Logical Operator11/1 -> [No_CAN4_BUS_OFF]
  Logical Operator12/1 -> [No_CAN_BUS_OFF]
  Logical Operator13/1 -> [No_CAN6_BUS_OFF]
  Logical Operator/1 -> Switch4/3
  Constant9/1 -> Switch4/2
  Constant6/1 -> Switch4/1
  Constant10/1 -> Switch5/1
  Constant14/1 -> Switch5/2
  Logical Operator2/1 -> Switch5/3
  Switch7/1 -> [VDDM_EDriveSysErrVCUErr_flg]  "VDDM_EDriveSysErrVCUErr_flg"
  Constant16/1 -> Equal1/2
  [VINP_DCDCFaultSta_enum] -> Equal1/1
  Data Type Conversion2/1 -> VDDM_HVRlyOpFail_flg/1  "VDDM_HVRlyOpFail_flg"
  Data Type Conversion3/1 -> VDDM_MCUActDisFail_flg/1  "VDDM_MCUActDisFail_flg"
  Data Type Conversion15/1 -> VDDM_VCUBrkSWSta_enum/1  "VDDM_VCUBrkSWSta_enum"
  Data Type Conversion4/1 -> VDDM_VCUFLDoorSta_flg/1  "VDDM_VCUFLDoorSta_flg"
  Data Type Conversion5/1 -> VDDM_VCUFRDoorSta_flg/1  "VDDM_VCUFRDoorSta_flg"
  Data Type Conversion6/1 -> VDDM_VCURLDoorSta_flg/1  "VDDM_VCURLDoorSta_flg"
  Data Type Conversion7/1 -> VDDM_VCURRDoorSta_flg/1  "VDDM_VCURRDoorSta_flg"
  Data Type Conversion8/1 -> VDDM_SysAllowReadySta_flg/1  "VDDM_SysAllowReadySta_flg"
  Data Type Conversion9/1 -> VDDM_VCUHoodSWSta_flg/1  "VDDM_VCUHoodSWSta_flg"
  Data Type Conversion10/1 -> VDDM_VCUTailgateSWSta_flg/1  "VDDM_VCUTailgateSWSta_flg"
  Data Type Conversion11/1 -> VDDM_EPB1NoComCFS_flg/1  "VDDM_EPB1NoComCFS_flg"
  Data Type Conversion12/1 -> VDDM_EPB1RCErrCFS_flg/1  "VDDM_EPB1RCErrCFS_flg"
  Data Type Conversion13/1 -> VDDM_EPB1CSErrCFS_flg/1  "VDDM_EPB1CSErrCFS_flg"
  Data Type Conversion14/1 -> VDDM_EPBSigErrCFS_flg/1  "VDDM_EPBSigErrCFS_flg"
  Ground4/1 -> Data Type Conversion2/1
  Ground22/1 -> Data Type Conversion3/1
  Ground24/1 -> Data Type Conversion15/1
  Ground23/1 -> Data Type Conversion4/1
  Ground28/1 -> Data Type Conversion5/1
  Ground25/1 -> Data Type Conversion6/1
  Ground27/1 -> Data Type Conversion7/1
  Ground26/1 -> Data Type Conversion8/1
  Ground36/1 -> Data Type Conversion9/1
  Ground29/1 -> Data Type Conversion10/1
  Ground31/1 -> Data Type Conversion11/1
  Ground30/1 -> Data Type Conversion12/1
  Ground35/1 -> Data Type Conversion13/1
  Ground32/1 -> Data Type Conversion14/1
  [VDDM_VehMalfunLevelTmp_enum] -> Relational Operator4/1
  Constant17/1 -> Relational Operator4/2
  Constant21/1 -> Switch7/3
  Constant18/1 -> Switch7/2
  Data Type Conversion/1 -> Switch7/1
  Constant19/1 -> Switch8/2
  Constant22/1 -> Switch8/3
  Switch2/1 -> Switch8/1
  Constant23/1 -> Switch9/2
  Constant24/1 -> Switch9/3
  Equal1/1 -> Switch9/1
  VINP_CAN1BusError_flg/1 -> [VINP_CAN1BusError_flg]
  VINP_CAN2BusError_flg/1 -> [VINP_CAN2BusError_flg]
  VINP_CAN3BusError_flg/1 -> [VINP_CAN3BusError_flg]
  VINP_CAN6BusError_flg/1 -> [VINP_CAN6BusError_flg]
  VINP_CAN5BusError_flg/1 -> [VINP_CAN5BusError_flg]
  VINP_CAN4BusError_flg/1 -> [VINP_CAN4BusError_flg]
  [VINP_CAN1BusError_flg] -> Subsystem/1(VINP_CAN1BusError_flg)
  [VINP_CAN6BusError_flg] -> Subsystem/6(VINP_CAN6BusError_flg)
  [VINP_CAN2BusError_flg] -> Subsystem/2(VINP_CAN2BusError_flg)
  [VINP_CAN3BusError_flg] -> Subsystem/3(VINP_CAN3BusError_flg)
  [VINP_CAN4BusError_flg] -> Subsystem/4(VINP_CAN4BusError_flg)
  [VINP_CAN5BusError_flg] -> Subsystem/5(VINP_CAN5BusError_flg)
  Subsystem/3(VDDM_CAN3BusErrorDTC_raw32) -> [VDDM_CAN3BusErrorDTC_raw32]
  Subsystem/2(VDDM_CAN2BusErrorDTC_raw32) -> [VDDM_CAN2BusErrorDTC_raw32]
  Subsystem/4(VDDM_CAN4BusErrorDTC_raw32) -> [VDDM_CAN4BusErrorDTC_raw32]
  Subsystem/1(VDDM_CAN1BusErrorDTC_raw32) -> [VDDM_CAN1BusErrorDTC_raw32]
  Subsystem/5(VDDM_CAN5BusErrorDTC_raw32) -> [VDDM_CAN5BusErrorDTC_raw32]
  Subsystem/6(VDDM_CAN6BusErrorDTC_raw32) -> [VDDM_CAN6BusErrorDTC_raw32]
  [VPMM_PwrStaSW_enum] -> Subsystem/7(VPMM_SysPwrSta_enum)
  [DTC_clear_request] -> Subsystem/8(DTC_clear_request)
  [VDDM_CAN4BusErrorDTC_raw32] -> VDDM_CAN4BusErrorDTC_raw32/1
  [VDDM_CAN2BusErrorDTC_raw32] -> VDDM_CAN2BusErrorDTC_raw32/1
  [VDDM_CAN5BusErrorDTC_raw32] -> VDDM_CAN5BusErrorDTC_raw32/1
  [VDDM_CAN3BusErrorDTC_raw32] -> VDDM_CAN3BusErrorDTC_raw32/1
  [VDDM_CAN6BusErrorDTC_raw32] -> VDDM_CAN6BusErrorDTC_raw32/1
  [VDDM_CAN1BusErrorDTC_raw32] -> VDDM_CAN1BusErrorDTC_raw32/1
